simulink library "pne_pne3d_generic_std"  (R2016a)
(part 6 of 7)

p510 "pne_brk_PowerBoost_massfracH2O (init) export=true name=pne_brk_PowerBoost_massfracH2O prio=1 dataSetName=std dataClassType=initIO dataClassName=initIO unit='-' description='pne_brk_PowerBoost_massfracH2O (init)': IO_PNE_Generic.pne_brk_PowerBoost_massfracH2O_0 [-]"; p511 "pne_brk_PowerBoost_mdot (init) export=true name=pne_brk_PowerBoost_mdot prio=1 dataSetName=std dataClassType=initIO dataClassName=initIO unit=kg/s description='pne_brk_PowerBoost_mdot': IO_PNE_Generic.pne_brk_PowerBoost_mdot_0 [-]"; p512 "pne_brk_PowerBoost_pressure [mbar] (init) export=true name=pne_brk_PowerBoost_pressure prio=1 dataSetName=std dataClassType=initIO dataClassName=initIO unit=mbar description='pne_brk_PowerBoost_pressure [mbar] (init)': IO_PNE_Generic.pne_brk_PowerBoost_pressure_0 [-]"; p513 "pne_brk_PowerBoost_Temperature [degC] (init) export=true name=pne_brk_PowerBoost_Temperature prio=1 dataSetName=std dataClassType=initIO dataClassName=initIO unit=degC description='pne_brk_PowerBoost_Temperature [degC] (init)': IO_PNE_Generic.pne_brk_PowerBoost_Temperature_0 [-]"; p514 "Parking Brake Pressure [bar] (init) export=true name=pne_brk_pRelPkBrk prio=1 dataSetName=std dataClassType=initIO dataClassName=initIO unit=bar description='Parking Brake Pressure [bar] (init)': IO_PNE_Generic.pne_brk_pRelPkBrk_0 [-]"; p515 "pne_brk_RearAxle_left_pAct (init) export=true name=pne_brk_RearAxle_left_pAct prio=1 dataSetName=std dataClassType=initIO dataClassName=initIO unit=bar description='pne_brk_RearAxle_left_pAct (init)': IO_PNE_Generic.pne_brk_RearAxle_left_pAct_0 [-]"; p516 "pne_brk_RearAxle_left_rotVel (init) export=true name=pne_brk_RearAxle_left_rotVel prio=1 dataSetName=std dataClassType=initIO dataClassName=initIO unit=rad/s description='pne_brk_RearAxle_left_rotVel (init)': IO_PNE_Generic.pne_brk_RearAxle_left_rotVel_0 [-]"; p517 "pne_brk_RearAxle_right_pAct (init) export=true name=pne_brk_RearAxle_right_pAct prio=1 dataSetName=std dataClassType=initIO dataClassName=initIO unit=bar description='pne_brk_RearAxle_right_pAct (init)': IO_PNE_Generic.pne_brk_RearAxle_right_pAct_0 [-]"; p518 "pne_brk_RearAxle_right_rotVel (init) export=true name=pne_brk_RearAxle_right_rotVel prio=1 dataSetName=std dataClassType=initIO dataClassName=initIO unit=rad/s description='pne_brk_RearAxle_right_rotVel (init)': IO_PNE_Generic.pne_brk_RearAxle_right_rotVel_0 [-]"; p519 "pne_brk_reg_active (init), Regeneraaton active export=true name=pne_brk_reg_active prio=1 dataSetName=std dataClassType=initIO dataClassName=initIO unit='-' description='Regeneraaton active': IO_PNE_Generic.pne_brk_reg_active_0 [-]"; p520 "wheel speed addional left wheel (init) export=true name=pne_brk_rotVel_al prio=1 dataSetName=std dataClassType=initIO dataClassName=initIO unit=rad/s description='wheel speed addional left wheel (init)': IO_PNE_Generic.pne_brk_rotVel_al_0 [-]"; p521 "wheel speed additional right wheel (init) export=true name=pne_brk_rotVel_ar prio=1 dataSetName=std dataClassType=initIO dataClassName=initIO unit=rad/s description='wheel speed additional right wheel (init)': IO_PNE_Generic.pne_brk_rotVel_ar_0 [-]"; p522 "wheel speed front left wheel (init) export=true name=pne_brk_rotVel_fl prio=1 dataSetName=std dataClassType=initIO dataClassName=initIO unit=rad/s description='wheel speed front left wheel (init)': IO_PNE_Generic.pne_brk_rotVel_fl_0 [-]"; p523 "wheel speed front right wheel (init) export=true name=pne_brk_rotVel_fr prio=1 dataSetName=std dataClassType=initIO dataClassName=initIO unit=rad/s description='wheel speed front right wheel (init)': IO_PNE_Generic.pne_brk_rotVel_fr_0 [-]"; p524 "wheel speed rear left wheel (init) export=true name=pne_brk_rotVel_rl prio=1 dataSetName=std dataClassType=initIO dataClassName=initIO unit=rad/s description='wheel speed rear left wheel (init)': IO_PNE_Generic.pne_brk_rotVel_rl_0 [-]"; p525 "wheel speed rear right wheel (init) export=true name=pne_brk_rotVel_rr prio=1 dataSetName=std dataClassType=initIO dataClassName=initIO unit=rad/s description='wheel speed rear right wheel (init)': IO_PNE_Generic.pne_brk_rotVel_rr_0 [-]"; p526 "wheel speed trailer axle1 left wheel (init) export=true name=pne_brk_rotVel_t1l prio=1 dataSetName=std dataClassType=initIO dataClassName=initIO unit=rad/s description='wheel speed trailer axle1 left wheel (init)': IO_PNE_Generic.pne_brk_rotVel_t1l_0 [-]"; p527 "wheel speed trailer axle1 right wheel (init) export=true name=pne_brk_rotVel_t1r prio=1 dataSetName=std dataClassType=initIO dataClassName=initIO unit=rad/s description='wheel speed trailer axle1 right wheel (init)': IO_PNE_Generic.pne_brk_rotVel_t1r_0 [-]"; p528 "wheel speed trailer axle2 left wheel (init) export=true name=pne_brk_rotVel_t2l prio=1 dataSetName=std dataClassType=initIO dataClassName=initIO unit=rad/s description='wheel speed trailer axle2 left wheel (init)': IO_PNE_Generic.pne_brk_rotVel_t2l_0 [-]"; p529 "wheel speed trailer axle2 right wheel (init) export=true name=pne_brk_rotVel_t2r prio=1 dataSetName=std dataClassType=initIO dataClassName=initIO unit=rad/s description='wheel speed trailer axle2 right wheel (init)': IO_PNE_Generic.pne_brk_rotVel_t2r_0 [-]"; p530 "wheel speed trailer axle3 left wheel (init) export=true name=pne_brk_rotVel_t3l prio=1 dataSetName=std dataClassType=initIO dataClassName=initIO unit=rad/s description='wheel speed trailer axle3 left wheel (init)': IO_PNE_Generic.pne_brk_rotVel_t3l_0 [-]"; p531 "wheel speed trailer axle3 right wheel (init) export=true name=pne_brk_rotVel_t3r prio=1 dataSetName=std dataClassType=initIO dataClassName=initIO unit=rad/s description='wheel speed trailer axle3 right wheel (init)': IO_PNE_Generic.pne_brk_rotVel_t3r_0 [-]"; p532 "pne_brk_TCV_pAct (init) export=true name=pne_brk_TCV_pAct prio=1 dataSetName=std dataClassType=initIO dataClassName=initIO unit=bar description='pne_brk_TCV_pAct (init)': IO_PNE_Generic.pne_brk_TCV_pAct_0 [-]"; p533 "pne_brk_Trailer_RV_Front_pAct (init) export=true name=pne_brk_Trailer_RV_Front_pAct prio=1 dataSetName=std dataClassType=initIO dataClassName=initIO unit=bar description='pne_brk_Trailer_RV_Front_pAct (init)': IO_PNE_Generic.pne_brk_Trailer_RV_Front_pAct_0 [-]"; p534 "pne_brk_Trailer_RV_Rear_pAct (init) export=true name=pne_brk_Trailer_RV_Rear_pAct prio=1 dataSetName=std dataClassType=initIO dataClassName=initIO unit=bar description='pne_brk_Trailer_RV_Rear_pAct (init)': IO_PNE_Generic.pne_brk_Trailer_RV_Rear_pAct_0 [-]"; p535 "pne_brk_TrailerAxle1_BrakingForce_at8p5bar [N] (init) export=true name=pne_brk_TrailerAxle1_BrakingForce_at8p5bar prio=1 dataSetName=std dataClassType=initIO dataClassName=initIO unit=N description='pne_brk_TrailerAxle1_BrakingForce_at8p5bar [N] (init)': IO_PNE_Generic.pne_brk_TrailerAxle1_BrakingForce_at8p5bar_0 [-]"; p536 "pne_brk_TrailerAxle1_BrakingPower [kW] (init) export=true name=pne_brk_TrailerAxle1_BrakingPower prio=1 dataSetName=std dataClassType=initIO dataClassName=initIO unit=kW description='pne_brk_TrailerAxle1_BrakingPower [kW] (init)': IO_PNE_Generic.pne_brk_TrailerAxle1_BrakingPower_0 [-]"; p537 "TrailerAxle 1 left - angular acceleration (init) export=true name=pne_brk_TrailerAxle1_left_angAcc prio=1 dataSetName=std dataClassType=initIO dataClassName=initIO unit=rad/s^2 description='TrailerAxle 1 left - angular acceleration (init)': IO_PNE_Generic.pne_brk_TrailerAxle1_left_angAcc_0 [-]"; p538 "Axle 1 left - angular position (init) export=true name=pne_brk_TrailerAxle1_left_angPos prio=1 dataSetName=std dataClassType=initIO dataClassName=initIO unit=bar description='TrailerAxle 1 left - angular position (init)': IO_PNE_Generic.pne_brk_TrailerAxle1_left_angPos_0 [-]"; p539 "Axle 1 left - angular velocity (init) export=true name=pne_brk_TrailerAxle1_left_angVel prio=1 dataSetName=std dataClassType=initIO dataClassName=initIO unit=rad/s description='TrailerAxle 1 left - angular velocity (init)': IO_PNE_Generic.pne_brk_TrailerAxle1_left_angVel_0 [-]"; p540 "brake correction coefficient kvT trailer axle 1 left (init) export=true name=pne_brk_TrailerAxle1_left_kvT prio=1 dataSetName=std dataClassType=initIO dataClassName=initIO unit='-' description='brake correction coefficient kvT trailer axle 1 left (init)': IO_PNE_Generic.pne_brk_TrailerAxle1_left_kvT_0 [-]"; p541 "brake pad thickness trailer axle 1 left (init) export=true name=pne_brk_TrailerAxle1_left_sPad_sum prio=1 dataSetName=std dataClassType=initIO dataClassName=initIO unit=m description='brake pad thickness trailer axle 1 left (init)': IO_PNE_Generic.pne_brk_TrailerAxle1_left_sPad_sum_0 [-]"; p542 "trailer axle 1 left temperature of the cooling surface area [degC] (init) export=true name=pne_brk_TrailerAxle1_left_Tcooldown prio=1 dataSetName=std dataClassType=initIO dataClassName=initIO unit=degC description='trailer axle 1 left temperature of the cooling surface area [degC] (init)': IO_PNE_Generic.pne_brk_TrailerAxle1_left_Tcooldown_0 [-]"; p543 "trailer axle 1 left temperature of the friction area [degC] (init) export=true name=pne_brk_TrailerAxle1_left_Tfriction prio=1 dataSetName=std dataClassType=initIO dataClassName=initIO unit=degC description='trailer axle 1 left temperature of the friction area [degC] (init)': IO_PNE_Generic.pne_brk_TrailerAxle1_left_Tfriction_0 [-]"; p544 "trailer axle 1 left temperature of the friction area [degC] (init) export=true name=pne_brk_TrailerAxle1_left_Tinterior prio=1 dataSetName=std dataClassType=initIO dataClassName=initIO unit=degC description='trailer axle 1 left inner temperature [degC] (init)': IO_PNE_Generic.pne_brk_TrailerAxle1_left_Tinterior_0 [-]"; p545 "pne_brk_TrailerAxle1_left_torque [Nm] (init) export=true name=pne_brk_TrailerAxle1_left_torque prio=1 dataSetName=std dataClassType=initIO dataClassName=initIO unit=Nm description='pne_brk_TrailerAxle1_left_torque [Nm] (init)': IO_PNE_Generic.pne_brk_TrailerAxle1_left_torque_0 [-]"; p546 "pne_brk_TrailerAxle1_left_torque_grinding [Nm] (init) export=true name=pne_brk_TrailerAxle1_left_torque_grinding prio=1 dataSetName=std dataClassType=initIO dataClassName=initIO unit=Nm description='pne_brk_TrailerAxle1_left_torque_grinding [Nm] (init)': IO_PNE_Generic.pne_brk_TrailerAxle1_left_torque_grinding_0 [-]"; p547 "TrailerAxle 1 right - angular acceleration (init) export=true name=pne_brk_TrailerAxle1_right_angAcc prio=1 dataSetName=std dataClassType=initIO dataClassName=initIO unit=rad/s^2 description='TrailerAxle 1 right - angular acceleration (init)': IO_PNE_Generic.pne_brk_TrailerAxle1_right_angAcc_0 [-]"; p548 "Axle 1 right - angular position (init) export=true name=pne_brk_TrailerAxle1_right_angPos prio=1 dataSetName=std dataClassType=initIO dataClassName=initIO unit=bar description='TrailerAxle 1 right - angular position (init)': IO_PNE_Generic.pne_brk_TrailerAxle1_right_angPos_0 [-]"; p549 "Axle 1 right - angular velocity (init) export=true name=pne_brk_TrailerAxle1_right_angVel prio=1 dataSetName=std dataClassType=initIO dataClassName=initIO unit=rad/s description='TrailerAxle 1 right - angular velocity (init)': IO_PNE_Generic.pne_brk_TrailerAxle1_right_angVel_0 [-]"; p550 "brake correction coefficient kvT trailer axle 1 right (init) export=true name=pne_brk_TrailerAxle1_right_kvT prio=1 dataSetName=std dataClassType=initIO dataClassName=initIO unit='-' description='brake correction coefficient kvT trailer axle 1 right (init)': IO_PNE_Generic.pne_brk_TrailerAxle1_right_kvT_0 [-]"; p551 "brake pad thickness trailer axle 1 right (init) export=true name=pne_brk_TrailerAxle1_right_sPad_sum prio=1 dataSetName=std dataClassType=initIO dataClassName=initIO unit=m description='brake pad thickness trailer axle 1 right (init)': IO_PNE_Generic.pne_brk_TrailerAxle1_right_sPad_sum_0 [-]"; p552 "trailer axle 1 right temperature of the cooling surface area [degC] (init) export=true name=pne_brk_TrailerAxle1_right_Tcooldown prio=1 dataSetName=std dataClassType=initIO dataClassName=initIO unit=degC description='trailer axle 1 right temperature of the cooling surface area [degC] (init)': IO_PNE_Generic.pne_brk_TrailerAxle1_right_Tcooldown_0 [-]"; p553 "trailer axle 1 right temperature of the friction area [degC] (init) export=true name=pne_brk_TrailerAxle1_right_Tfriction prio=1 dataSetName=std dataClassType=initIO dataClassName=initIO unit=degC description='trailer axle 1 right temperature of the friction area [degC] (init)': IO_PNE_Generic.pne_brk_TrailerAxle1_right_Tfriction_0 [-]"; p554 "trailer axle 1 right temperature of the friction area [degC] (init) export=true name=pne_brk_TrailerAxle1_right_Tinterior prio=1 dataSetName=std dataClassType=initIO dataClassName=initIO unit=degC description='trailer axle 1 right inner temperature [degC] (init)': IO_PNE_Generic.pne_brk_TrailerAxle1_right_Tinterior_0 [-]"; p555 "pne_brk_TrailerAxle1_right_torque [Nm] (init) export=true name=pne_brk_TrailerAxle1_right_torque prio=1 dataSetName=std dataClassType=initIO dataClassName=initIO unit=Nm description='pne_brk_TrailerAxle1_right_torque [Nm] (init)': IO_PNE_Generic.pne_brk_TrailerAxle1_right_torque_0 [-]"; p556 "pne_brk_TrailerAxle1_right_torque_grinding [Nm] (init) export=true name=pne_brk_TrailerAxle1_right_torque_grinding prio=1 dataSetName=std dataClassType=initIO dataClassName=initIO unit=Nm description='pne_brk_TrailerAxle1_right_torque_grinding [Nm] (init)': IO_PNE_Generic.pne_brk_TrailerAxle1_right_torque_grinding_0 [-]"; p557 "pne_brk_TrailerAxle1_torque_sns [Nm] (init) export=true name=pne_brk_TrailerAxle1_torque_sns prio=1 dataSetName=std dataClassType=initIO dataClassName=initIO unit=Nm description='pne_brk_TrailerAxle1_torque_sns [Nm] (init)': IO_PNE_Generic.pne_brk_TrailerAxle1_torque_sns_0 [-]"; p558 "Cylinder Force Trailer Brake Cylinder1 [N] (init) export=true name=pne_brk_TrailerAxle1Brake_Fcyl prio=1 dataSetName=std dataClassType=initIO dataClassName=initIO unit=N description='Cylinder Force Trailer Brake Cylinder1 [N] (init)': IO_PNE_Generic.pne_brk_TrailerAxle1Brake_Fcyl_0 [-]"; p559 "Pressure (relative) Trailer Brake Cylinder1 left [bar] (init) export=true name=pne_brk_TrailerAxle1Brake_left_pRel prio=1 dataSetName=std dataClassType=initIO dataClassName=initIO unit=bar description='Pressure (relative) Trailer Brake Cylinder1 left [bar] (init)': IO_PNE_Generic.pne_brk_TrailerAxle1Brake_left_pRel_0 [-]"; p560 "Pressure (relative) Trailer Brake Cylinder1 right [bar] (init) export=true name=pne_brk_TrailerAxle1Brake_right_pRel prio=1 dataSetName=std dataClassType=initIO dataClassName=initIO unit=bar description='Pressure (relative) Trailer Brake Cylinder1 right [bar] (init)': IO_PNE_Generic.pne_brk_TrailerAxle1Brake_right_pRel_0 [-]"; p561 "Piston Stroke Trailer Brake Cylinder1 [mm] (init) export=true name=pne_brk_TrailerAxle1Brake_stroke prio=1 dataSetName=std dataClassType=initIO dataClassName=initIO unit=mm description='Piston Stroke Trailer Brake Cylinder1 [mm] (init)': IO_PNE_Generic.pne_brk_TrailerAxle1Brake_stroke_0 [-]"; p562 "pne_brk_TrailerAxle1Brake_Vol [dm3] (init) export=true name=pne_brk_TrailerAxle1Brake_Vol prio=1 dataSetName=std dataClassType=initIO dataClassName=initIO unit=l description='pne_brk_TrailerAxle1Brake_Vol [dm3] (init)': IO_PNE_Generic.pne_brk_TrailerAxle1Brake_Vol_0 [-]"; p563 "pne_brk_TrailerAxle2_BrakingForce_at8p5bar [N] (init) export=true name=pne_brk_TrailerAxle2_BrakingForce_at8p5bar prio=1 dataSetName=std dataClassType=initIO dataClassName=initIO unit=N description='pne_brk_TrailerAxle2_BrakingForce_at8p5bar [N] (init)': IO_PNE_Generic.pne_brk_TrailerAxle2_BrakingForce_at8p5bar_0 [-]"; p564 "pne_brk_TrailerAxle2_BrakingPower [kW] (init) export=true name=pne_brk_TrailerAxle2_BrakingPower prio=1 dataSetName=std dataClassType=initIO dataClassName=initIO unit=kW description='pne_brk_TrailerAxle2_BrakingPower [kW] (init)': IO_PNE_Generic.pne_brk_TrailerAxle2_BrakingPower_0 [-]"; p565 "TrailerAxle 2 left - angular acceleration (init) export=true name=pne_brk_TrailerAxle2_left_angAcc prio=1 dataSetName=std dataClassType=initIO dataClassName=initIO unit=rad/s^2 description='TrailerAxle 2 left - angular acceleration (init)': IO_PNE_Generic.pne_brk_TrailerAxle2_left_angAcc_0 [-]"; p566 "TrailerAxle 2 left - angular position (init) export=true name=pne_brk_TrailerAxle2_left_angPos prio=1 dataSetName=std dataClassType=initIO dataClassName=initIO unit=bar description='TrailerAxle 2 left - angular position (init)': IO_PNE_Generic.pne_brk_TrailerAxle2_left_angPos_0 [-]"; p567 "TrailerAxle 2 left - angular velocity (init) export=true name=pne_brk_TrailerAxle2_left_angVel prio=1 dataSetName=std dataClassType=initIO dataClassName=initIO unit=rad/s description='TrailerAxle 2 left - angular velocity (init)': IO_PNE_Generic.pne_brk_TrailerAxle2_left_angVel_0 [-]"; p568 "brake correction coefficient kvT trailer axle 2 left (init) export=true name=pne_brk_TrailerAxle2_left_kvT prio=1 dataSetName=std dataClassType=initIO dataClassName=initIO unit='-' description='brake correction coefficient kvT trailer axle 2 left (init)': IO_PNE_Generic.pne_brk_TrailerAxle2_left_kvT_0 [-]"; p569 "brake pad thickness trailer axle 2 left (init) export=true name=pne_brk_TrailerAxle2_left_sPad_sum prio=1 dataSetName=std dataClassType=initIO dataClassName=initIO unit=m description='brake pad thickness trailer axle 2 left (init)': IO_PNE_Generic.pne_brk_TrailerAxle2_left_sPad_sum_0 [-]"; p570 "trailer axle 2 left temperature of the cooling surface area [degC] (init) export=true name=pne_brk_TrailerAxle2_left_Tcooldown prio=1 dataSetName=std dataClassType=initIO dataClassName=initIO unit=degC description='trailer axle 2 left temperature of the cooling surface area [degC] (init)': IO_PNE_Generic.pne_brk_TrailerAxle2_left_Tcooldown_0 [-]"; p571 "trailer axle 2 left temperature of the friction area [degC] (init) export=true name=pne_brk_TrailerAxle2_left_Tfriction prio=1 dataSetName=std dataClassType=initIO dataClassName=initIO unit=degC description='trailer axle 2 left temperature of the friction area [degC] (init)': IO_PNE_Generic.pne_brk_TrailerAxle2_left_Tfriction_0 [-]"; p572 "trailer axle 2 left temperature of the friction area [degC] (init) export=true name=pne_brk_TrailerAxle2_left_Tinterior prio=1 dataSetName=std dataClassType=initIO dataClassName=initIO unit=degC description='trailer axle 2 left inner temperature [degC] (init)': IO_PNE_Generic.pne_brk_TrailerAxle2_left_Tinterior_0 [-]"; p573 "pne_brk_TrailerAxle2_left_torque [Nm] (init) export=true name=pne_brk_TrailerAxle2_left_torque prio=1 dataSetName=std dataClassType=initIO dataClassName=initIO unit=Nm description='pne_brk_TrailerAxle2_left_torque [Nm] (init)': IO_PNE_Generic.pne_brk_TrailerAxle2_left_torque_0 [-]"; p574 "pne_brk_TrailerAxle2_left_torque_grinding [Nm] (init) export=true name=pne_brk_TrailerAxle2_left_torque_grinding prio=1 dataSetName=std dataClassType=initIO dataClassName=initIO unit=Nm description='pne_brk_TrailerAxle2_left_torque_grinding [Nm] (init)': IO_PNE_Generic.pne_brk_TrailerAxle2_left_torque_grinding_0 [-]"; p575 "TrailerAxle 2 right - angular acceleration (init) export=true name=pne_brk_TrailerAxle2_right_angAcc prio=1 dataSetName=std dataClassType=initIO dataClassName=initIO unit=rad/s^2 description='TrailerAxle 2 right - angular acceleration (init)': IO_PNE_Generic.pne_brk_TrailerAxle2_right_angAcc_0 [-]"; p576 "TrailerAxle 2 right - angular position (init) export=true name=pne_brk_TrailerAxle2_right_angPos prio=1 dataSetName=std dataClassType=initIO dataClassName=initIO unit=bar description='TrailerAxle 2 right - angular position (init)': IO_PNE_Generic.pne_brk_TrailerAxle2_right_angPos_0 [-]"; p577 "TrailerAxle 2 right - angular velocity (init) export=true name=pne_brk_TrailerAxle2_right_angVel prio=1 dataSetName=std dataClassType=initIO dataClassName=initIO unit=rad/s description='TrailerAxle 2 right - angular velocity (init)': IO_PNE_Generic.pne_brk_TrailerAxle2_right_angVel_0 [-]"; p578 "brake correction coefficient kvT trailer axle 2 right (init) export=true name=pne_brk_TrailerAxle2_right_kvT prio=1 dataSetName=std dataClassType=initIO dataClassName=initIO unit='-' description='brake correction coefficient kvT trailer axle 2 right (init)': IO_PNE_Generic.pne_brk_TrailerAxle2_right_kvT_0 [-]"; p579 "brake pad thickness trailer axle 2 right (init) export=true name=pne_brk_TrailerAxle2_right_sPad_sum prio=1 dataSetName=std dataClassType=initIO dataClassName=initIO unit=m description='brake pad thickness trailer axle 2 right (init)': IO_PNE_Generic.pne_brk_TrailerAxle2_right_sPad_sum_0 [-]"; p580 "trailer axle 2 right temperature of the cooling surface area [degC] (init) export=true name=pne_brk_TrailerAxle2_right_Tcooldown prio=1 dataSetName=std dataClassType=initIO dataClassName=initIO unit=degC description='trailer axle 2 right temperature of the cooling surface area [degC] (init)': IO_PNE_Generic.pne_brk_TrailerAxle2_right_Tcooldown_0 [-]"; p581 "trailer axle 2 right temperature of the friction area [degC] (init) export=true name=pne_brk_TrailerAxle2_right_Tfriction prio=1 dataSetName=std dataClassType=initIO dataClassName=initIO unit=degC description='trailer axle 2 right temperature of the friction area [degC] (init)': IO_PNE_Generic.pne_brk_TrailerAxle2_right_Tfriction_0 [-]"; p582 "trailer axle 2 right temperature of the friction area [degC] (init) export=true name=pne_brk_TrailerAxle2_right_Tinterior prio=1 dataSetName=std dataClassType=initIO dataClassName=initIO unit=degC description='trailer axle 2 right inner temperature [degC] (init)': IO_PNE_Generic.pne_brk_TrailerAxle2_right_Tinterior_0 [-]"; p583 "pne_brk_TrailerAxle2_right_torque [Nm] (init) export=true name=pne_brk_TrailerAxle2_right_torque prio=1 dataSetName=std dataClassType=initIO dataClassName=initIO unit=Nm description='pne_brk_TrailerAxle2_right_torque [Nm] (init)': IO_PNE_Generic.pne_brk_TrailerAxle2_right_torque_0 [-]"; p584 "pne_brk_TrailerAxle2_right_torque_grinding [Nm] (init) export=true name=pne_brk_TrailerAxle2_right_torque_grinding prio=1 dataSetName=std dataClassType=initIO dataClassName=initIO unit=Nm description='pne_brk_TrailerAxle2_right_torque_grinding [Nm] (init)': IO_PNE_Generic.pne_brk_TrailerAxle2_right_torque_grinding_0 [-]"; p585 "pne_brk_TrailerAxle2_torque_sns [Nm] (init) export=true name=pne_brk_TrailerAxle2_torque_sns prio=1 dataSetName=std dataClassType=initIO dataClassName=initIO unit=Nm description='pne_brk_TrailerAxle2_torque_sns [Nm] (init)': IO_PNE_Generic.pne_brk_TrailerAxle2_torque_sns_0 [-]"; p586 "Cylinder Force Trailer Brake Cylinder2 [N] (init) export=true name=pne_brk_TrailerAxle2Brake_Fcyl prio=1 dataSetName=std dataClassType=initIO dataClassName=initIO unit=N description='Cylinder Force Trailer Brake Cylinder2 [N] (init)': IO_PNE_Generic.pne_brk_TrailerAxle2Brake_Fcyl_0 [-]"; p587 "Pressure (relative) Trailer Brake Cylinder2 left [bar] (init) export=true name=pne_brk_TrailerAxle2Brake_left_pRel prio=1 dataSetName=std dataClassType=initIO dataClassName=initIO unit=bar description='Pressure (relative) Trailer Brake Cylinder2 left [bar] (init)': IO_PNE_Generic.pne_brk_TrailerAxle2Brake_left_pRel_0 [-]"; p588 "Pressure (relative) Trailer Brake Cylinder2 right [bar] (init) export=true name=pne_brk_TrailerAxle2Brake_right_pRel prio=1 dataSetName=std dataClassType=initIO dataClassName=initIO unit=bar description='Pressure (relative) Trailer Brake Cylinder2 right [bar] (init)': IO_PNE_Generic.pne_brk_TrailerAxle2Brake_right_pRel_0 [-]"; p589 "Piston Stroke Trailer Brake Cylinder2 [mm] (init) export=true name=pne_brk_TrailerAxle2Brake_stroke prio=1 dataSetName=std dataClassType=initIO dataClassName=initIO unit=mm description='Piston Stroke Trailer Brake Cylinder2 [mm] (init)': IO_PNE_Generic.pne_brk_TrailerAxle2Brake_stroke_0 [-]"; p590 "pne_brk_TrailerAxle2Brake_Vol [dm3] (init) export=true name=pne_brk_TrailerAxle2Brake_Vol prio=1 dataSetName=std dataClassType=initIO dataClassName=initIO unit=l description='pne_brk_TrailerAxle2Brake_Vol [dm3] (init)': IO_PNE_Generic.pne_brk_TrailerAxle2Brake_Vol_0 [-]"; p591 "pne_brk_TrailerAxle3_BrakingForce_at8p5bar [N] (init) export=true name=pne_brk_TrailerAxle3_BrakingForce_at8p5bar prio=1 dataSetName=std dataClassType=initIO dataClassName=initIO unit=N description='pne_brk_TrailerAxle3_BrakingForce_at8p5bar [N] (init)': IO_PNE_Generic.pne_brk_TrailerAxle3_BrakingForce_at8p5bar_0 [-]"; p592 "pne_brk_TrailerAxle3_BrakingPower [kW] (init) export=true name=pne_brk_TrailerAxle3_BrakingPower prio=1 dataSetName=std dataClassType=initIO dataClassName=initIO unit=kW description='pne_brk_TrailerAxle3_BrakingPower [kW] (init)': IO_PNE_Generic.pne_brk_TrailerAxle3_BrakingPower_0 [-]"; p593 "TrailerAxle 3 left - angular acceleration (init) export=true name=pne_brk_TrailerAxle3_left_angAcc prio=1 dataSetName=std dataClassType=initIO dataClassName=initIO unit=rad/s^2 description='TrailerAxle 3 left - angular acceleration (init)': IO_PNE_Generic.pne_brk_TrailerAxle3_left_angAcc_0 [-]"; p594 "TrailerAxle 3 left - angular position (init) export=true name=pne_brk_TrailerAxle3_left_angPos prio=1 dataSetName=std dataClassType=initIO dataClassName=initIO unit=bar description='TrailerAxle 3 left - angular position (init)': IO_PNE_Generic.pne_brk_TrailerAxle3_left_angPos_0 [-]"; p595 "TrailerAxle 3 left - angular velocity (init) export=true name=pne_brk_TrailerAxle3_left_angVel prio=1 dataSetName=std dataClassType=initIO dataClassName=initIO unit=rad/s description='TrailerAxle 3 left - angular velocity (init)': IO_PNE_Generic.pne_brk_TrailerAxle3_left_angVel_0 [-]"; p596 "brake correction coefficient kvT trailer axle 3 left (init) export=true name=pne_brk_TrailerAxle3_left_kvT prio=1 dataSetName=std dataClassType=initIO dataClassName=initIO unit='-' description='brake correction coefficient kvT trailer axle 3 left (init)': IO_PNE_Generic.pne_brk_TrailerAxle3_left_kvT_0 [-]"; p597 "brake pad thickness trailer axle 3 left (init) export=true name=pne_brk_TrailerAxle3_left_sPad_sum prio=1 dataSetName=std dataClassType=initIO dataClassName=initIO unit=m description='brake pad thickness trailer axle 3 left (init)': IO_PNE_Generic.pne_brk_TrailerAxle3_left_sPad_sum_0 [-]"; p598 "trailer axle 3 left temperature of the cooling surface area [degC] (init) export=true name=pne_brk_TrailerAxle3_left_Tcooldown prio=1 dataSetName=std dataClassType=initIO dataClassName=initIO unit=degC description='trailer axle 3 left temperature of the cooling surface area [degC] (init)': IO_PNE_Generic.pne_brk_TrailerAxle3_left_Tcooldown_0 [-]"; p599 "trailer axle 3 left temperature of the friction area [degC] (init) export=true name=pne_brk_TrailerAxle3_left_Tfriction prio=1 dataSetName=std dataClassType=initIO dataClassName=initIO unit=degC description='trailer axle 3 left temperature of the friction area [degC] (init)': IO_PNE_Generic.pne_brk_TrailerAxle3_left_Tfriction_0 [-]"; p600 "trailer axle 3 left temperature of the friction area [degC] (init) export=true name=pne_brk_TrailerAxle3_left_Tinterior prio=1 dataSetName=std dataClassType=initIO dataClassName=initIO unit=degC description='trailer axle 3 left inner temperature [degC] (init)': IO_PNE_Generic.pne_brk_TrailerAxle3_left_Tinterior_0 [-]"; p601 "pne_brk_TrailerAxle3_left_torque [Nm] (init) export=true name=pne_brk_TrailerAxle3_left_torque prio=1 dataSetName=std dataClassType=initIO dataClassName=initIO unit=Nm description='pne_brk_TrailerAxle3_left_torque [Nm] (init)': IO_PNE_Generic.pne_brk_TrailerAxle3_left_torque_0 [-]"; p602 "pne_brk_TrailerAxle3_left_torque_grinding [Nm] (init) export=true name=pne_brk_TrailerAxle3_left_torque_grinding prio=1 dataSetName=std dataClassType=initIO dataClassName=initIO unit=Nm description='pne_brk_TrailerAxle3_left_torque_grinding [Nm] (init)': IO_PNE_Generic.pne_brk_TrailerAxle3_left_torque_grinding_0 [-]"; p603 "TrailerAxle 3 right - angular acceleration (init) export=true name=pne_brk_TrailerAxle3_right_angAcc prio=1 dataSetName=std dataClassType=initIO dataClassName=initIO unit=rad/s^2 description='TrailerAxle 3 right - angular acceleration (init)': IO_PNE_Generic.pne_brk_TrailerAxle3_right_angAcc_0 [-]"; p604 "TrailerAxle 3 right - angular position (init) export=true name=pne_brk_TrailerAxle3_right_angPos prio=1 dataSetName=std dataClassType=initIO dataClassName=initIO unit=bar description='TrailerAxle 3 right - angular position (init)': IO_PNE_Generic.pne_brk_TrailerAxle3_right_angPos_0 [-]"; p605 "TrailerAxle 3 right - angular velocity (init) export=true name=pne_brk_TrailerAxle3_right_angVel prio=1 dataSetName=std dataClassType=initIO dataClassName=initIO unit=rad/s description='TrailerAxle 3 right - angular velocity (init)': IO_PNE_Generic.pne_brk_TrailerAxle3_right_angVel_0 [-]"; p606 "brake correction coefficient kvT trailer axle 3 right (init) export=true name=pne_brk_TrailerAxle3_right_kvT prio=1 dataSetName=std dataClassType=initIO dataClassName=initIO unit='-' description='brake correction coefficient kvT trailer axle 3 right (init)': IO_PNE_Generic.pne_brk_TrailerAxle3_right_kvT_0 [-]"; p607 "brake pad thickness trailer axle 3 right (init) export=true name=pne_brk_TrailerAxle3_right_sPad_sum prio=1 dataSetName=std dataClassType=initIO dataClassName=initIO unit=m description='brake pad thickness trailer axle 3 right (init)': IO_PNE_Generic.pne_brk_TrailerAxle3_right_sPad_sum_0 [-]"; p608 "trailer axle 3 right temperature of the cooling surface area [degC] (init) export=true name=pne_brk_TrailerAxle3_right_Tcooldown prio=1 dataSetName=std dataClassType=initIO dataClassName=initIO unit=degC description='trailer axle 3 right temperature of the cooling surface area [degC] (init)': IO_PNE_Generic.pne_brk_TrailerAxle3_right_Tcooldown_0 [-]"; p609 "trailer axle 3 right temperature of the friction area [degC] (init) export=true name=pne_brk_TrailerAxle3_right_Tfriction prio=1 dataSetName=std dataClassType=initIO dataClassName=initIO unit=degC description='trailer axle 3 right temperature of the friction area [degC] (init)': IO_PNE_Generic.pne_brk_TrailerAxle3_right_Tfriction_0 [-]"; p610 "trailer axle 3 right temperature of the friction area [degC] (init) export=true name=pne_brk_TrailerAxle3_right_Tinterior prio=1 dataSetName=std dataClassType=initIO dataClassName=initIO unit=degC description='trailer axle 3 right inner temperature [degC] (init)': IO_PNE_Generic.pne_brk_TrailerAxle3_right_Tinterior_0 [-]"; p611 "pne_brk_TrailerAxle3_right_torque [Nm] (init) export=true name=pne_brk_TrailerAxle3_right_torque prio=1 dataSetName=std dataClassType=initIO dataClassName=initIO unit=Nm description='pne_brk_TrailerAxle3_right_torque [Nm] (init)': IO_PNE_Generic.pne_brk_TrailerAxle3_right_torque_0 [-]"; p612 "pne_brk_TrailerAxle3_right_torque_grinding [Nm] (init) export=true name=pne_brk_TrailerAxle3_right_torque_grinding prio=1 dataSetName=std dataClassType=initIO dataClassName=initIO unit=Nm description='pne_brk_TrailerAxle3_right_torque_grinding [Nm] (init)': IO_PNE_Generic.pne_brk_TrailerAxle3_right_torque_grinding_0 [-]"; p613 "pne_brk_TrailerAxle3_torque_sns [Nm] (init) export=true name=pne_brk_TrailerAxle3_torque_sns prio=1 dataSetName=std dataClassType=initIO dataClassName=initIO unit=Nm description='pne_brk_TrailerAxle3_torque_sns [Nm] (init)': IO_PNE_Generic.pne_brk_TrailerAxle3_torque_sns_0 [-]"; p614 "Cylinder Force Trailer Brake Cylinder3 [N] (init) export=true name=pne_brk_TrailerAxle3Brake_Fcyl prio=1 dataSetName=std dataClassType=initIO dataClassName=initIO unit=N description='Cylinder Force Trailer Brake Cylinder3 [N] (init)': IO_PNE_Generic.pne_brk_TrailerAxle3Brake_Fcyl_0 [-]"; p615 "Pressure (relative) Trailer Brake Cylinder3 left [bar] (init) export=true name=pne_brk_TrailerAxle3Brake_left_pRel prio=1 dataSetName=std dataClassType=initIO dataClassName=initIO unit=bar description='Pressure (relative) Trailer Brake Cylinder3 left [bar] (init)': IO_PNE_Generic.pne_brk_TrailerAxle3Brake_left_pRel_0 [-]"; p616 "Pressure (relative) Trailer Brake Cylinder3 right [bar] (init) export=true name=pne_brk_TrailerAxle3Brake_right_pRel prio=1 dataSetName=std dataClassType=initIO dataClassName=initIO unit=bar description='Pressure (relative) Trailer Brake Cylinder3 right [bar] (init)': IO_PNE_Generic.pne_brk_TrailerAxle3Brake_right_pRel_0 [-]"; p617 "Piston Stroke Trailer Brake Cylinder3 [mm] (init) export=true name=pne_brk_TrailerAxle3Brake_stroke prio=1 dataSetName=std dataClassType=initIO dataClassName=initIO unit=mm description='Piston Stroke Trailer Brake Cylinder3 [mm] (init)': IO_PNE_Generic.pne_brk_TrailerAxle3Brake_stroke_0 [-]"; p618 "pne_brk_TrailerAxle3Brake_Vol [dm^3] (init) export=true name=pne_brk_TrailerAxle3Brake_Vol prio=1 dataSetName=std dataClassType=initIO dataClassName=initIO unit=l description='pne_brk_TrailerAxle3Brake_Vol [dm^3] (init)': IO_PNE_Generic.pne_brk_TrailerAxle3Brake_Vol_0 [-]"; p619 "Relative Pressure Tank1 [bar] (init) export=true name=pne_brk_V1_pRel prio=1 dataSetName=std dataClassType=initIO dataClassName=initIO unit=bar description='Relative Pressure Tank1 [bar] (init) ': IO_PNE_Generic.pne_brk_V1_pRel_0 [-]"; p620 "Temperature Tank1 [degC] (init) export=true name=pne_brk_V1_Temp prio=1 dataSetName=std dataClassType=initIO dataClassName=initIO unit=degC description='Temperature Tank1 [degC] (init)': IO_PNE_Generic.pne_brk_V1_Temp_0 [-]"; p621 "Relative Pressure Tank2 [bar] (init) export=true name=pne_brk_V2_pRel prio=1 dataSetName=std dataClassType=initIO dataClassName=initIO unit=bar description='Relative Pressure Tank2 [bar] (init) ': IO_PNE_Generic.pne_brk_V2_pRel_0 [-]"; p622 "Temperature Tank2 [degC] (init) export=true name=pne_brk_V2_Temp prio=1 dataSetName=std dataClassType=initIO dataClassName=initIO unit=degC description='Temperature Tank2 [degC] (init)': IO_PNE_Generic.pne_brk_V2_Temp_0 [-]"; p623 "Relative Pressure Tank3 [bar] (init) export=true name=pne_brk_V3_pRel prio=1 dataSetName=std dataClassType=initIO dataClassName=initIO unit=bar description='Relative Pressure Tank3 [bar] (init)': IO_PNE_Generic.pne_brk_V3_pRel_0 [-]"; p624 "Temperature Tank3 [degC] (init) export=true name=pne_brk_V3_Temp prio=1 dataSetName=std dataClassType=initIO dataClassName=initIO unit=degC description='Temperature Tank3 [degC] (init)': IO_PNE_Generic.pne_brk_V3_Temp_0 [-]"; p625 "Relative Pressure Tank4 [bar] (init) export=true name=pne_brk_V4_pRel prio=1 dataSetName=std dataClassType=initIO dataClassName=initIO unit=bar description='Relative Pressure Tank4 [bar] (init)': IO_PNE_Generic.pne_brk_V4_pRel_0 [-]"; p626 "Temperature Tank4 [degC] (init) export=true name=pne_brk_V4_Temp prio=1 dataSetName=std dataClassType=initIO dataClassName=initIO unit=degC description='Temperature Tank4 [degC] (init)': IO_PNE_Generic.pne_brk_V4_Temp_0 [-]"; p627 "Relative Pressure Tank5 [bar] (init) export=true name=pne_brk_V5_pRel prio=1 dataSetName=std dataClassType=initIO dataClassName=initIO unit=bar description='Relative Pressure Tank5 [bar] (init)': IO_PNE_Generic.pne_brk_V5_pRel_0 [-]"; p628 "Temperature Tank5 [degC] (init) export=true name=pne_brk_V5_Temp prio=1 dataSetName=std dataClassType=initIO dataClassName=initIO unit=degC description='Temperature Tank5 [degC] (init)': IO_PNE_Generic.pne_brk_V5_Temp_0 [-]"; p629 "Relative Pressure Tank6 [bar] (init) export=true name=pne_brk_V6_pRel prio=1 dataSetName=std dataClassType=initIO dataClassName=initIO unit=bar description='Relative Pressure Tank6 [bar] (init)': IO_PNE_Generic.pne_brk_V6_pRel_0 [-]"; p630 "Temperature Tank6 [degC] (init) export=true name=pne_brk_V6_Temp prio=1 dataSetName=std dataClassType=initIO dataClassName=initIO unit=degC description='Temperature Tank6 [degC] (init)': IO_PNE_Generic.pne_brk_V6_Temp_0 [-]"; p631 "Relative Pressure Tank7 [bar] (init) export=true name=pne_brk_V7_pRel prio=1 dataSetName=std dataClassType=initIO dataClassName=initIO unit=bar description='Relative Pressure Tank7 [bar] (init)': IO_PNE_Generic.pne_brk_V7_pRel_0 [-]"; p632 "Temperature Tank7 [degC] (init) export=true name=pne_brk_V7_Temp prio=1 dataSetName=std dataClassType=initIO dataClassName=initIO unit=degC description='Temperature Tank7 [degC] (init)': IO_PNE_Generic.pne_brk_V7_Temp_0 [-]"; p633 "Relative Pressure Tank8 [bar] (init) export=true name=pne_brk_V8_pRel prio=1 dataSetName=std dataClassType=initIO dataClassName=initIO unit=bar description='Relative Pressure Tank8 [bar] (init)': IO_PNE_Generic.pne_brk_V8_pRel_0 [-]"; p634 "Temperature Tank8 [degC] (init) export=true name=pne_brk_V8_Temp prio=1 dataSetName=std dataClassType=initIO dataClassName=initIO unit=degC description='Temperature Tank8 [degC] (init)': IO_PNE_Generic.pne_brk_V8_Temp_0 [-]"; p635 "Relative Pressure Vsupply Input [bar] (init) export=true name=pne_brk_Vsup_pRel prio=1 dataSetName=std dataClassType=initIO dataClassName=initIO unit=bar description='Relative Pressure Vsupply Input [bar] (init)': IO_PNE_Generic.pne_brk_Vsup_pRel_0 [-]"; p636 "Temperature Vsupply Input [degC] (init) export=true name=pne_brk_Vsup_Temp prio=1 dataSetName=std dataClassType=initIO dataClassName=initIO unit=degC description='Temperature Vsupply Input [degC] (init)': IO_PNE_Generic.pne_brk_Vsup_Temp_0 [-]"; p637 "Relative Pressure Tank Trailer [bar] (init) export=true name=pne_brk_VTrailer_pRel prio=1 dataSetName=std dataClassType=initIO dataClassName=initIO unit=bar description='Relative Pressure Tank Trailer [bar] (init)': IO_PNE_Generic.pne_brk_VTrailer_pRel_0 [-]"; p638 "Temperature Tank Trailer [degC] (init) export=true name=pne_brk_VTrailer_Temp prio=1 dataSetName=std dataClassType=initIO dataClassName=initIO unit=degC description='Temperature Tank Trailer [degC] (init)': IO_PNE_Generic.pne_brk_VTrailer_Temp_0 [-]"; p639 "pne_brk_WetLvl_Cntr (init), Calculated Wettnesslevel of the cartridge / Nl export=true name=pne_brk_WetLvl_Cntr prio=1 dataSetName=std dataClassType=initIO dataClassName=initIO unit='Nl' description='Calculated Wettnesslevel of the cartridge / Nl': IO_PNE_Generic.pne_brk_WetLvl_Cntr_0 [-]"; p640 "pne_susp_A1_Le_Posn (init) export=true name=pne_susp_A1_Le_Posn prio=1 dataSetName=std dataClassType=initIO dataClassName=initIO unit='-' description='pne_susp_A1_Le_Posn (init)': IO_PNE_Generic.pne_susp_A1_Le_Posn_0 [-]"; p641 "pne_susp_A1_Ri_Posn (init) export=true name=pne_susp_A1_Ri_Posn prio=1 dataSetName=std dataClassType=initIO dataClassName=initIO unit='-' description='pne_susp_A1_Ri_Posn (init)': IO_PNE_Generic.pne_susp_A1_Ri_Posn_0 [-]"; p642 "pne_susp_A2_Le_Posn (init) export=true name=pne_susp_A2_Le_Posn prio=1 dataSetName=std dataClassType=initIO dataClassName=initIO unit='-' description='pne_susp_A2_Le_Posn (init)': IO_PNE_Generic.pne_susp_A2_Le_Posn_0 [-]"; p643 "pne_susp_A2_Ri_Posn (init) export=true name=pne_susp_A2_Ri_Posn prio=1 dataSetName=std dataClassType=initIO dataClassName=initIO unit='-' description='pne_susp_A2_Ri_Posn (init)': IO_PNE_Generic.pne_susp_A2_Ri_Posn_0 [-]"; p644 "pne_susp_A3_Le_Posn (init) export=true name=pne_susp_A3_Le_Posn prio=1 dataSetName=std dataClassType=initIO dataClassName=initIO unit='-' description='pne_susp_A3_Le_Posn (init)': IO_PNE_Generic.pne_susp_A3_Le_Posn_0 [-]"; p645 "pne_susp_A3_Ri_Posn (init) export=true name=pne_susp_A3_Ri_Posn prio=1 dataSetName=std dataClassType=initIO dataClassName=initIO unit='-' description='pne_susp_A3_Ri_Posn (init)': IO_PNE_Generic.pne_susp_A3_Ri_Posn_0 [-]"; p646 "pneAux_A1_Le_Rq (init) export=true name=pneAux_A1_Le_Rq prio=1 dataSetName=std dataClassType=initIO dataClassName=initIO unit='-' description='pneAux_A1_Le_Rq': IO_PNE_Generic.pneAux_A1_Le_Rq_0 [-]"; p647 "pneAux_A1_LoLi_Rq (init) export=true name=pneAux_A1_LoLi_Rq prio=1 dataSetName=std dataClassType=initIO dataClassName=initIO unit='-' description='pneAux_A1_LoLi_Rq': IO_PNE_Generic.pneAux_A1_LoLi_Rq_0 [-]"; p648 "pneAux_A1_Ri_Rq (init) export=true name=pneAux_A1_Ri_Rq prio=1 dataSetName=std dataClassType=initIO dataClassName=initIO unit='-' description='pneAux_A1_Ri_Rq': IO_PNE_Generic.pneAux_A1_Ri_Rq_0 [-]"; p649 "pneAux_A2_Le_Rq (init) export=true name=pneAux_A2_Le_Rq prio=1 dataSetName=std dataClassType=initIO dataClassName=initIO unit='-' description='pneAux_A2_Le_Rq': IO_PNE_Generic.pneAux_A2_Le_Rq_0 [-]"; p650 "pneAux_A2_LoLi_Rq (init) export=true name=pneAux_A2_LoLi_Rq prio=1 dataSetName=std dataClassType=initIO dataClassName=initIO unit='-' description='pneAux_A2_LoLi_Rq': IO_PNE_Generic.pneAux_A2_LoLi_Rq_0 [-]"; p651 "pneAux_A2_Ri_Rq (init) export=true name=pneAux_A2_Ri_Rq prio=1 dataSetName=std dataClassType=initIO dataClassName=initIO unit='-' description='pneAux_A2_Ri_Rq': IO_PNE_Generic.pneAux_A2_Ri_Rq_0 [-]"; p652 "pneAux_A3_Le_Rq (init) export=true name=pneAux_A3_Le_Rq prio=1 dataSetName=std dataClassType=initIO dataClassName=initIO unit='-' description='pneAux_A3_Le_Rq': IO_PNE_Generic.pneAux_A3_Le_Rq_0 [-]"; p653 "pneAux_A3_LoLi_Rq (init) export=true name=pneAux_A3_LoLi_Rq prio=1 dataSetName=std dataClassType=initIO dataClassName=initIO unit='-' description='pneAux_A3_LoLi_Rq': IO_PNE_Generic.pneAux_A3_LoLi_Rq_0 [-]"; p654 "pneAux_A3_Ri_Rq (init) export=true name=pneAux_A3_Ri_Rq prio=1 dataSetName=std dataClassType=initIO dataClassName=initIO unit='-' description='pneAux_A3_Ri_Rq (init)': IO_PNE_Generic.pneAux_A3_Ri_Rq_0 [-]"; p655 "pneAux_Axle1_load (init) export=true name=pneAux_Axle1_load prio=1 dataSetName=std dataClassType=initIO dataClassName=initIO unit=kg description='pneAux_Axle1_load': IO_PNE_Generic.pneAux_Axle1_load_0 [-]"; p656 "pneAux_Axle2_load (init) export=true name=pneAux_Axle2_load prio=1 dataSetName=std dataClassType=initIO dataClassName=initIO unit=kg description='pneAux_Axle2_load': IO_PNE_Generic.pneAux_Axle2_load_0 [-]"; p657 "pneAux_Axle3_load (init) export=true name=pneAux_Axle3_load prio=1 dataSetName=std dataClassType=initIO dataClassName=initIO unit=kg description='pneAux_Axle3_load': IO_PNE_Generic.pneAux_Axle3_load_0 [-]"; p658 "pneAux_Axle4_load (init) export=true name=pneAux_Axle4_load prio=1 dataSetName=std dataClassType=initIO dataClassName=initIO unit=kg description='pneAux_Axle4_load': IO_PNE_Generic.pneAux_Axle4_load_0 [-]"; p659 "pneAux_Drs_Rq (init) export=true name=pneAux_Drs_Rq prio=1 dataSetName=std dataClassType=initIO dataClassName=initIO unit='-' description='pneAux_Drs_Rq': IO_PNE_Generic.pneAux_Drs_Rq_0 [-]"; p660 "pneAux_EAPU_overrun (init) export=true name=pneAux_EAPU_overrun prio=1 dataSetName=std dataClassType=initIO dataClassName=initIO unit='-' description='pneAux_EAPU_overrun': IO_PNE_Generic.pneAux_EAPU_overrun_0 [-]"; p661 "pneAux_pSoll_TCV_p43 Trailer Parking Brake (init) export=true name=pneAux_pSoll_TCV_p43 prio=1 dataSetName=std dataClassType=initIO dataClassName=initIO unit=bar description='pneAux_pSoll_TCV_p43 Trailer Parking Brake (init)': IO_PNE_Generic.pneAux_pSoll_TCV_p43_0 [-]"; p662 "Set Pressure Parking Brake (init) export=true name=pneAux_pSollPkBrk prio=1 dataSetName=std dataClassType=initIO dataClassName=initIO unit=bar description='Set Pressure Parking Brake (init)': IO_PNE_Generic.pneAux_pSollPkBrk_0 [-]"; p663 "pneAux_TCV_pDmd_Front_Left (init) export=true name=pneAux_TCV_pDmd_Front_Left prio=1 dataSetName=std dataClassType=initIO dataClassName=initIO unit='-' description='pneAux_TCV_pDmd_Front_Left': IO_PNE_Generic.pneAux_TCV_pDmd_Front_Left_0 [-]"; p664 "pneAux_TCV_pDmd_Front_Right (init) export=true name=pneAux_TCV_pDmd_Front_Right prio=1 dataSetName=std dataClassType=initIO dataClassName=initIO unit='-' description='pneAux_TCV_pDmd_Front_Right': IO_PNE_Generic.pneAux_TCV_pDmd_Front_Right_0 [-]"; p665 "pneAux_TCV_pDmd_Rear_Left (init) export=true name=pneAux_TCV_pDmd_Rear_Left prio=1 dataSetName=std dataClassType=initIO dataClassName=initIO unit='-' description='pneAux_TCV_pDmd_Rear_Left': IO_PNE_Generic.pneAux_TCV_pDmd_Rear_Left_0 [-]"; p666 "pneAux_TCV_pDmd_Rear_Right (init) export=true name=pneAux_TCV_pDmd_Rear_Right prio=1 dataSetName=std dataClassType=initIO dataClassName=initIO unit='-' description='pneAux_TCV_pDmd_Rear_Right': IO_PNE_Generic.pneAux_TCV_pDmd_Rear_Right_0 [-]"; p667 "pneAux_trailerAxle1_left_stABSInValve (init) export=true name=pneAux_trailerAxle1_left_stABSInValve prio=1 dataSetName=std dataClassType=initIO dataClassName=initIO unit='-' description='pneAux_trailerAxle1_left_stABSInValve': IO_PNE_Generic.pneAux_trailerAxle1_left_stABSInValve_0 [-]"; p668 "pneAux_trailerAxle1_left_stABSOutValve (init) export=true name=pneAux_trailerAxle1_left_stABSOutValve prio=1 dataSetName=std dataClassType=initIO dataClassName=initIO unit='-' description='pneAux_trailerAxle1_left_stABSOutValve': IO_PNE_Generic.pneAux_trailerAxle1_left_stABSOutValve_0 [-]"; p669 "pneAux_trailerAxle1_load (init) export=true name=pneAux_trailerAxle1_load prio=1 dataSetName=std dataClassType=initIO dataClassName=initIO unit=kg description='pneAux_trailerAxle1_load': IO_PNE_Generic.pneAux_trailerAxle1_load_0 [-]"; p670 "pneAux_trailerAxle1_right_stABSInValve (init) export=true name=pneAux_trailerAxle1_right_stABSInValve prio=1 dataSetName=std dataClassType=initIO dataClassName=initIO unit='-' description='pneAux_trailerAxle1_right_stABSInValve': IO_PNE_Generic.pneAux_trailerAxle1_right_stABSInValve_0 [-]"; p671 "pneAux_trailerAxle1_right_stABSOutValve (init) export=true name=pneAux_trailerAxle1_right_stABSOutValve prio=1 dataSetName=std dataClassType=initIO dataClassName=initIO unit='-' description='pneAux_trailerAxle1_right_stABSOutValve': IO_PNE_Generic.pneAux_trailerAxle1_right_stABSOutValve_0 [-]"; p672 "pneAux_trailerAxle2_left_stABSInValve (init) export=true name=pneAux_trailerAxle2_left_stABSInValve prio=1 dataSetName=std dataClassType=initIO dataClassName=initIO unit='-' description='pneAux_trailerAxle2_left_stABSInValve': IO_PNE_Generic.pneAux_trailerAxle2_left_stABSInValve_0 [-]"; p673 "pneAux_trailerAxle2_left_stABSOutValve (init) export=true name=pneAux_trailerAxle2_left_stABSOutValve prio=1 dataSetName=std dataClassType=initIO dataClassName=initIO unit='-' description='pneAux_trailerAxle2_left_stABSOutValve': IO_PNE_Generic.pneAux_trailerAxle2_left_stABSOutValve_0 [-]"; p674 "pneAux_trailerAxle2_load (init) export=true name=pneAux_trailerAxle2_load prio=1 dataSetName=std dataClassType=initIO dataClassName=initIO unit=kg description='pneAux_trailerAxle2_load': IO_PNE_Generic.pneAux_trailerAxle2_load_0 [-]"; p675 "pneAux_trailerAxle2_right_stABSInValve (init) export=true name=pneAux_trailerAxle2_right_stABSInValve prio=1 dataSetName=std dataClassType=initIO dataClassName=initIO unit='-' description='pneAux_trailerAxle2_right_stABSInValve': IO_PNE_Generic.pneAux_trailerAxle2_right_stABSInValve_0 [-]"; p676 "pneAux_trailerAxle2_right_stABSOutValve (init) export=true name=pneAux_trailerAxle2_right_stABSOutValve prio=1 dataSetName=std dataClassType=initIO dataClassName=initIO unit='-' description='pneAux_trailerAxle2_right_stABSOutValve': IO_PNE_Generic.pneAux_trailerAxle2_right_stABSOutValve_0 [-]"; p677 "pneAux_trailerAxle3_left_stABSInValve (init) export=true name=pneAux_trailerAxle3_left_stABSInValve prio=1 dataSetName=std dataClassType=initIO dataClassName=initIO unit='-' description='pneAux_trailerAxle3_left_stABSInValve': IO_PNE_Generic.pneAux_trailerAxle3_left_stABSInValve_0 [-]"; p678 "pneAux_trailerAxle3_left_stABSOutValve (init) export=true name=pneAux_trailerAxle3_left_stABSOutValve prio=1 dataSetName=std dataClassType=initIO dataClassName=initIO unit='-' description='pneAux_trailerAxle3_left_stABSOutValve': IO_PNE_Generic.pneAux_trailerAxle3_left_stABSOutValve_0 [-]"; p679 "pneAux_trailerAxle3_load (init) export=true name=pneAux_trailerAxle3_load prio=1 dataSetName=std dataClassType=initIO dataClassName=initIO unit=kg description='pneAux_trailerAxle3_load': IO_PNE_Generic.pneAux_trailerAxle3_load_0 [-]"; p680 "pneAux_trailerAxle3_right_stABSInValve (init) export=true name=pneAux_trailerAxle3_right_stABSInValve prio=1 dataSetName=std dataClassType=initIO dataClassName=initIO unit='-' description='pneAux_trailerAxle3_right_stABSInValve': IO_PNE_Generic.pneAux_trailerAxle3_right_stABSInValve_0 [-]"; p681 "pneAux_trailerAxle3_right_stABSOutValve (init) export=true name=pneAux_trailerAxle3_right_stABSOutValve prio=1 dataSetName=std dataClassType=initIO dataClassName=initIO unit='-' description='pneAux_trailerAxle3_right_stABSOutValve': IO_PNE_Generic.pneAux_trailerAxle3_right_stABSOutValve_0 [-]"; p682 "Leakage Nominal Flow [l/min] export=true name=QnLeak prio=1 dataSetName=auxil_dummy dataClassType=auxil dataClassName=auxil unit='l' description='Leakage Nominal Flow [l/min]': leakageQn.QnLeak [-]"; p683 "step Size [s] export=true name=stepSize prio=1 dataSetName=veh_dummy dataClassType=veh dataClassName=veh unit='s' description=' step size [s]': pne3d_veh_Param.stepSize [s]"; p684 "Time Constant for Outlet Pressure Build Up APCV export=true name=T1_APCV prio=1 dataSetName=veh_dummy dataClassType=veh dataClassName=veh unit=s description='Time Constant for Outlet Pressure Build Up APCV': pne3d_veh_Param.T1_APCV [s]"; p685 "Time Constant for Outlet Pressure Build Up CMAX export=true name=T1_CMAX prio=1 dataSetName=veh_dummy dataClassType=veh dataClassName=veh unit=s description='Time Constant for Outlet Pressure Build Up CMAX': pne3d_veh_Param.T1_CMAX [s]"; p686 "Compressor Inlet Temperature Offset [K] export=true name=dT_CompInlet prio=1 dataSetName=pro_dummy dataClassType=pro dataClassName=pro unit='K' description='Compressor Inlet Temperature Offset [K]': pneumaticsParam.dT_CompInlet [-]"; p687 "US System Layout [0-false, 1-true,2-US6s6m] export=true name=flagUS prio=1 dataSetName=pro_dummy dataClassType=pro dataClassName=pro unit='-' description='US System Layout [0-false, 1-true,2-US6s6m]': pneumaticsParam.flagUS [-]"; p688 "Compressor Cut In Pressure (relative) at normal drive conditions [bar] export=true name=pRelCI prio=1 dataSetName=pro_dummy dataClassType=pro dataClassName=pro unit='bar' description='Compressor Cut In Pressure (relative) at normal drive conditions [bar]': pneumaticsParam.pRelCI [-]"; p689 "Compressor Cut In Pressure (relative) during Engine Run Over [bar] export=true name=pRelCI_RO prio=1 dataSetName=pro_dummy dataClassType=pro dataClassName=pro unit='bar' description='Compressor Cut In Pressure (relative) during Engine Run Over [bar]': pneumaticsParam.pRelCI_RO [-]"; p690 "Compressor Cut Off Pressure (relative) at normal drive conditions [bar] export=true name=pRelCO prio=1 dataSetName=pro_dummy dataClassType=pro dataClassName=pro unit='bar' description='Compressor Cut Off Pressure (relative) at normal drive conditions [bar]': pneumaticsParam.pRelCO [-]"; p691 "Compressor Cut Off Pressure (relative) during Engine Run Over [bar] export=true name=pRelCO_RO prio=1 dataSetName=pro_dummy dataClassType=pro dataClassName=pro unit='bar' description='Compressor Cut Off Pressure (relative) during Engine Run Over [bar]': pneumaticsParam.pRelCO_RO [-]"; p692 "EAPU Limitng Pressure (relative) primary circuits (V1, V2) [bar] export=true name=pRelLimit_C1C2 prio=1 dataSetName=pro_dummy dataClassType=pro dataClassName=pro unit='bar' description='EAPU Limitng Pressure (relative) primary circuits (V1, V2) [bar]': pneumaticsParam.pRelLimit_C1C2 [-]"; p693 "EAPU Limitng Pressure (relative) secondary circuits (V3, V4, V5, V6) [bar] export=true name=pRelLimit_C3C4 prio=1 dataSetName=pro_dummy dataClassType=pro dataClassName=pro unit='bar' description='EAPU Limitng Pressure (relative) secondary circuits (V3, V4, V5, V6) [bar]': pneumaticsParam.pRelLimit_C3C4 [-]"; p694 "EAPU Percentage of Regeneration [%] export=true name=RegenPct prio=1 dataSetName=pro_dummy dataClassType=pro dataClassName=pro unit='%' description='EAPU Percentage of Regeneration [%]': pneumaticsParam.RegenPct [-]"; p695 "Volume Tank1 [dm^3] export=true name=V1 prio=1 dataSetName=pro_dummy dataClassType=pro dataClassName=pro unit='dm^3' description='Volume Tank1 [dm^3]': pneumaticsParam.V1 [-]"; p696 "Volume Tank2 [dm^3] export=true name=V2 prio=1 dataSetName=pro_dummy dataClassType=pro dataClassName=pro unit='dm^3' description='Volume Tank2 [dm^3]': pneumaticsParam.V2 [-]"; p697 "Volume Tank3 [dm^3] export=true name=V3 prio=1 dataSetName=pro_dummy dataClassType=pro dataClassName=pro unit='dm^3' description='Volume Tank3 [dm^3]': pneumaticsParam.V3 [-]"; p698 "Volume Tank4 [dm^3] export=true name=V4 prio=1 dataSetName=pro_dummy dataClassType=pro dataClassName=pro unit='dm^3' description='Volume Tank4 [dm^3]': pneumaticsParam.V4 [-]"; p699 "Volume Tank5 [dm^3] export=true name=V5 prio=1 dataSetName=pro_dummy dataClassType=pro dataClassName=pro unit='dm^3' description='Volume Tank5 [dm^3]': pneumaticsParam.V5 [-]"; p700 "Volume Tank6 [dm^3] export=true name=V6 prio=1 dataSetName=pro_dummy dataClassType=pro dataClassName=pro unit='dm^3' description='Volume Tank6 [dm^3]': pneumaticsParam.V6 [-]"; p701 "Volume Tank7 [dm^3] export=true name=V7 prio=1 dataSetName=pro_dummy dataClassType=pro dataClassName=pro unit='dm^3' description='Volume Tank7 [dm^3]': pneumaticsParam.V7 [-]"; p702 "Volume Tank8 [dm^3] export=true name=V8 prio=1 dataSetName=pro_dummy dataClassType=pro dataClassName=pro unit='dm^3' description='Volume Tank8 [dm^3]': pneumaticsParam.V8 [-]"; p703 "Intake Volume of Cartridge [dm^3] export=true name=Vcartridge prio=1 dataSetName=pro_dummy dataClassType=pro dataClassName=pro unit='dm^3' description='Intake Volume of Cartridge [dm^3]': pneumaticsParam.Vcartridge [-]"; p704 "Intake Volume of Cooling Pipe [dm^3] export=true name=Vintake prio=1 dataSetName=pro_dummy dataClassType=pro dataClassName=pro unit='dm^3' description='Intake Volume of Cooling Pipe [dm^3]': pneumaticsParam.Vintake [-]"; p705 "Volume Tank Regeneration [dm^3] export=true name=Vreg prio=1 dataSetName=pro_dummy dataClassType=pro dataClassName=pro unit='dm^3' description='Volume Tank Regeneration [dm^3]': pneumaticsParam.Vreg [-]"; p706 "Volume Tank Supply [dm^3] export=true name=Vsup prio=1 dataSetName=pro_dummy dataClassType=pro dataClassName=pro unit='dm^3' description='Volume Tank Supply [dm^3]': pneumaticsParam.Vsup [-]"; p707 "SCR Nominal Flow [l/min] export=true name=QnSCR prio=1 dataSetName=auxil_dummy dataClassType=auxil dataClassName=auxil unit='l' description=SCR Nominal Flow [l/min]': SCR.QnSCR [-]"; p708 "temperatures calculation of brakes (0->No/1->Yes) export=true name=TemperatureCalculation prio=1 dataSetName=default dataClassType=initialTemperatures dataClassName=initialTemperatures unit='' description='temperatures calculation of brakes (0->No/1->Yes)': T_initial_brakes_Param.TemperatureCalculation [-]"; p709 "Air Consumption for Lifting of dxRef at Axle Load {mAxle, dV} [l] export=true name=dV_mAxle_Ref prio=1 dataSetName=susp_dummy dataClassType=susp dataClassName=$dataSetClassAirSpring$ unit='l' description='Air Consumption for Lifting of dxRef at Axle Load {mAxle, dV} [l]': airSpring_Axle1.dV_mAxle_Ref [-]"; p710 "Air Consumption for Lifting of dxRef at Axle Load {mAxle, dV} [l] export=true name=dV_mAxle_Ref prio=1 dataSetName=susp_dummy dataClassType=susp dataClassName=$dataSetClassAirSpring$ unit='l' description='Air Consumption for Lifting of dxRef at Axle Load {mAxle, dV} [l]': airSpring_Axle2.dV_mAxle_Ref [-]"; p711 "Air Consumption for Lifting of dxRef at Axle Load {mAxle, dV} [l] export=true name=dV_mAxle_Ref prio=1 dataSetName=susp_dummy dataClassType=susp dataClassName=$dataSetClassAirSpring$ unit='l' description='Air Consumption for Lifting of dxRef at Axle Load {mAxle, dV} [l]': airSpring_Axle3.dV_mAxle_Ref [-]"; p712 "Air Consumption for Lifting of dxRef at Axle Load {mAxle, dV} [l] export=true name=dV_mAxle_Ref prio=1 dataSetName=susp_dummy dataClassType=susp dataClassName=$dataSetClassAirSpring$ unit='l' description='Air Consumption for Lifting of dxRef at Axle Load {mAxle, dV} [l]': airSpring_Axle4.dV_mAxle_Ref [-]"; p713 "Temperature Values (x-Axis) of fac_T Temperature Correction Curve export=true name=fac_T_xAxis prio=1 dataSetName=brk_dummy dataClassType=brk dataClassName=$dataSetClassBrk$  unit='degC' description='Temperature Values in [degC] (x-Axis) of fac_T Temperature Correction Curve': BrakeA1_R.fac_T_xAxis [-]"; p714 "Correction Coefficient Values (y-Axis) of fac_T Temperature Correction Curve export=true name=fac_T_yAxis prio=1 dataSetName=brk_dummy dataClassType=brk dataClassName=$dataSetClassBrk$  unit='-' description='Correction Coefficient Values (y-Axis) of fac_T Temperature Correction Curve': BrakeA1_R.fac_T_yAxis [-]"; p715 "Velocity Values (x-Axis) of fac_v_Velocity Correction Curve export=true name=fac_v_xAxis prio=1 dataSetName=brk_dummy dataClassType=brk dataClassName=$dataSetClassBrk$  unit='m/s' description='Velocity Values (x-Axis) of fac_v_Velocity Correction Curve': BrakeA1_R.fac_v_xAxis [-]"; p716 "Correction Coefficient Values (y-Axis) of fac_v Temperature Correction Curve export=true name=fac_v_yAxis prio=1 dataSetName=brk_dummy dataClassType=brk dataClassName=$dataSetClassBrk$  unit='-' description='Correction Coefficient Values (y-Axis) of fac_v Velocity Correction Curve': BrakeA1_R.fac_v_yAxis [-]"; p717 "Force Values (x-Axis) of Lever Force-Displacement Curve export=true name=Fdx_xAxis prio=1 dataSetName=brk_dummy dataClassType=brk dataClassName=$dataSetClassBrk$  unit='N' description='Force Values (x-Axis) of Lever Force-Displacement Curve': BrakeA1_R.Fdx_xAxis [N]"; p718 "Displacement Values (y-Axis) of Lever Force-Displacement Curve export=true name=Fdx_yAxis prio=1 dataSetName=brk_dummy dataClassType=brk dataClassName=$dataSetClassBrk$  unit='m' description='Displacement Values (y-Axis) of Lever Force-Displacement Curve': BrakeA1_R.Fdx_yAxis [m]"; p719 "Displacement Values (x-Axis) of Lever Displacement-i Ratio Curve export=true name=i_xAxis prio=1 dataSetName=brk_dummy dataClassType=brk dataClassName=$dataSetClassBrk$  unit='m' description='Displacement Values (x-Axis) of Lever Displacement-i Ratio Curve': BrakeA1_R.i_xAxis [m]"; p720 "i Ratio Values (y-Axis) of Lever Displacement-i Ratio Curve export=true name=i_yAxis prio=1 dataSetName=brk_dummy dataClassType=brk dataClassName=$dataSetClassBrk$  unit='-' description='i Ratio Values (y-Axis) of Lever Displacement-i Ratio Curve': BrakeA1_R.i_yAxis [-]"; p721 "Temperature Values in [degC] (x-Axis) of wearRate-T-Curve export=true name=wearRate_T_xAxis prio=1 dataSetName=brk_dummy dataClassType=brk dataClassName=$dataSetClassBrk$  unit='degC' description='Temperature Values in [degC] (x-Axis) of wearRate-T-Curve': BrakeA1_R.wearRate_T_xAxis [-]"; p722 "Wear Rate Values (y-Axis) of wearRate-T-Curve [cm^3/kWh] export=true name=wearRate_T_yAxis prio=1 dataSetName=brk_dummy dataClassType=brk dataClassName=$dataSetClassBrk$  unit='-' description='Wear Rate Values (y-Axis) of wearRate-T-Curve [cm^3/kWh]': BrakeA1_R.wearRate_T_yAxis [-]"; p723 "Temperature Values (x-Axis) of fac_T Temperature Correction Curve export=true name=fac_T_xAxis prio=1 dataSetName=brk_dummy dataClassType=brk dataClassName=$dataSetClassBrk$  unit='degC' description='Temperature Values in [degC] (x-Axis) of fac_T Temperature Correction Curve': BrakeA2_R.fac_T_xAxis [-]"; p724 "Correction Coefficient Values (y-Axis) of fac_T Temperature Correction Curve export=true name=fac_T_yAxis prio=1 dataSetName=brk_dummy dataClassType=brk dataClassName=$dataSetClassBrk$  unit='-' description='Correction Coefficient Values (y-Axis) of fac_T Temperature Correction Curve': BrakeA2_R.fac_T_yAxis [-]"; p725 "Velocity Values (x-Axis) of fac_v_Velocity Correction Curve export=true name=fac_v_xAxis prio=1 dataSetName=brk_dummy dataClassType=brk dataClassName=$dataSetClassBrk$  unit='m/s' description='Velocity Values (x-Axis) of fac_v_Velocity Correction Curve': BrakeA2_R.fac_v_xAxis [-]"; p726 "Correction Coefficient Values (y-Axis) of fac_v Temperature Correction Curve export=true name=fac_v_yAxis prio=1 dataSetName=brk_dummy dataClassType=brk dataClassName=$dataSetClassBrk$  unit='-' description='Correction Coefficient Values (y-Axis) of fac_v Velocity Correction Curve': BrakeA2_R.fac_v_yAxis [-]"; p727 "Force Values (x-Axis) of Lever Force-Displacement Curve export=true name=Fdx_xAxis prio=1 dataSetName=brk_dummy dataClassType=brk dataClassName=$dataSetClassBrk$  unit='N' description='Force Values (x-Axis) of Lever Force-Displacement Curve': BrakeA2_R.Fdx_xAxis [N]"; p728 "Displacement Values (y-Axis) of Lever Force-Displacement Curve export=true name=Fdx_yAxis prio=1 dataSetName=brk_dummy dataClassType=brk dataClassName=$dataSetClassBrk$  unit='m' description='Displacement Values (y-Axis) of Lever Force-Displacement Curve': BrakeA2_R.Fdx_yAxis [m]"; p729 "Displacement Values (x-Axis) of Lever Displacement-i Ratio Curve export=true name=i_xAxis prio=1 dataSetName=brk_dummy dataClassType=brk dataClassName=$dataSetClassBrk$  unit='m' description='Displacement Values (x-Axis) of Lever Displacement-i Ratio Curve': BrakeA2_R.i_xAxis [m]"; p730 "i Ratio Values (y-Axis) of Lever Displacement-i Ratio Curve export=true name=i_yAxis prio=1 dataSetName=brk_dummy dataClassType=brk dataClassName=$dataSetClassBrk$  unit='-' description='i Ratio Values (y-Axis) of Lever Displacement-i Ratio Curve': BrakeA2_R.i_yAxis [-]"; p731 "Temperature Values in [degC] (x-Axis) of wearRate-T-Curve export=true name=wearRate_T_xAxis prio=1 dataSetName=brk_dummy dataClassType=brk dataClassName=$dataSetClassBrk$  unit='degC' description='Temperature Values in [degC] (x-Axis) of wearRate-T-Curve': BrakeA2_R.wearRate_T_xAxis [-]"; p732 "Wear Rate Values (y-Axis) of wearRate-T-Curve [cm^3/kWh] export=true name=wearRate_T_yAxis prio=1 dataSetName=brk_dummy dataClassType=brk dataClassName=$dataSetClassBrk$  unit='-' description='Wear Rate Values (y-Axis) of wearRate-T-Curve [cm^3/kWh]': BrakeA2_R.wearRate_T_yAxis [-]"; p733 "Temperature Values (x-Axis) of fac_T Temperature Correction Curve export=true name=fac_T_xAxis prio=1 dataSetName=brk_dummy dataClassType=brk dataClassName=$dataSetClassBrk$  unit='degC' description='Temperature Values in [degC] (x-Axis) of fac_T Temperature Correction Curve': BrakeA3_R.fac_T_xAxis [-]"; p734 "Correction Coefficient Values (y-Axis) of fac_T Temperature Correction Curve export=true name=fac_T_yAxis prio=1 dataSetName=brk_dummy dataClassType=brk dataClassName=$dataSetClassBrk$  unit='-' description='Correction Coefficient Values (y-Axis) of fac_T Temperature Correction Curve': BrakeA3_R.fac_T_yAxis [-]"; p735 "Velocity Values (x-Axis) of fac_v_Velocity Correction Curve export=true name=fac_v_xAxis prio=1 dataSetName=brk_dummy dataClassType=brk dataClassName=$dataSetClassBrk$  unit='m/s' description='Velocity Values (x-Axis) of fac_v_Velocity Correction Curve': BrakeA3_R.fac_v_xAxis [-]"; p736 "Correction Coefficient Values (y-Axis) of fac_v Temperature Correction Curve export=true name=fac_v_yAxis prio=1 dataSetName=brk_dummy dataClassType=brk dataClassName=$dataSetClassBrk$  unit='-' description='Correction Coefficient Values (y-Axis) of fac_v Velocity Correction Curve': BrakeA3_R.fac_v_yAxis [-]"; p737 "Force Values (x-Axis) of Lever Force-Displacement Curve export=true name=Fdx_xAxis prio=1 dataSetName=brk_dummy dataClassType=brk dataClassName=$dataSetClassBrk$  unit='N' description='Force Values (x-Axis) of Lever Force-Displacement Curve': BrakeA3_R.Fdx_xAxis [N]"; p738 "Displacement Values (y-Axis) of Lever Force-Displacement Curve export=true name=Fdx_yAxis prio=1 dataSetName=brk_dummy dataClassType=brk dataClassName=$dataSetClassBrk$  unit='m' description='Displacement Values (y-Axis) of Lever Force-Displacement Curve': BrakeA3_R.Fdx_yAxis [m]"; p739 "Displacement Values (x-Axis) of Lever Displacement-i Ratio Curve export=true name=i_xAxis prio=1 dataSetName=brk_dummy dataClassType=brk dataClassName=$dataSetClassBrk$  unit='m' description='Displacement Values (x-Axis) of Lever Displacement-i Ratio Curve': BrakeA3_R.i_xAxis [m]"; p740 "i Ratio Values (y-Axis) of Lever Displacement-i Ratio Curve export=true name=i_yAxis prio=1 dataSetName=brk_dummy dataClassType=brk dataClassName=$dataSetClassBrk$  unit='-' description='i Ratio Values (y-Axis) of Lever Displacement-i Ratio Curve': BrakeA3_R.i_yAxis [-]"; p741 "Temperature Values in [degC] (x-Axis) of wearRate-T-Curve export=true name=wearRate_T_xAxis prio=1 dataSetName=brk_dummy dataClassType=brk dataClassName=$dataSetClassBrk$  unit='degC' description='Temperature Values in [degC] (x-Axis) of wearRate-T-Curve': BrakeA3_R.wearRate_T_xAxis [-]"; p742 "Wear Rate Values (y-Axis) of wearRate-T-Curve [cm^3/kWh] export=true name=wearRate_T_yAxis prio=1 dataSetName=brk_dummy dataClassType=brk dataClassName=$dataSetClassBrk$  unit='-' description='Wear Rate Values (y-Axis) of wearRate-T-Curve [cm^3/kWh]': BrakeA3_R.wearRate_T_yAxis [-]"; p743 "Temperature Values (x-Axis) of fac_T Temperature Correction Curve export=true name=fac_T_xAxis prio=1 dataSetName=brk_dummy dataClassType=brk dataClassName=$dataSetClassBrk$  unit='degC' description='Temperature Values in [degC] (x-Axis) of fac_T Temperature Correction Curve': BrakeA4_R.fac_T_xAxis [-]"; p744 "Correction Coefficient Values (y-Axis) of fac_T Temperature Correction Curve export=true name=fac_T_yAxis prio=1 dataSetName=brk_dummy dataClassType=brk dataClassName=$dataSetClassBrk$  unit='-' description='Correction Coefficient Values (y-Axis) of fac_T Temperature Correction Curve': BrakeA4_R.fac_T_yAxis [-]"; p745 "Velocity Values (x-Axis) of fac_v_Velocity Correction Curve export=true name=fac_v_xAxis prio=1 dataSetName=brk_dummy dataClassType=brk dataClassName=$dataSetClassBrk$  unit='m/s' description='Velocity Values (x-Axis) of fac_v_Velocity Correction Curve': BrakeA4_R.fac_v_xAxis [-]"; p746 "Correction Coefficient Values (y-Axis) of fac_v Temperature Correction Curve export=true name=fac_v_yAxis prio=1 dataSetName=brk_dummy dataClassType=brk dataClassName=$dataSetClassBrk$  unit='-' description='Correction Coefficient Values (y-Axis) of fac_v Velocity Correction Curve': BrakeA4_R.fac_v_yAxis [-]"; p747 "Force Values (x-Axis) of Lever Force-Displacement Curve export=true name=Fdx_xAxis prio=1 dataSetName=brk_dummy dataClassType=brk dataClassName=$dataSetClassBrk$  unit='N' description='Force Values (x-Axis) of Lever Force-Displacement Curve': BrakeA4_R.Fdx_xAxis [N]"; p748 "Displacement Values (y-Axis) of Lever Force-Displacement Curve export=true name=Fdx_yAxis prio=1 dataSetName=brk_dummy dataClassType=brk dataClassName=$dataSetClassBrk$  unit='m' description='Displacement Values (y-Axis) of Lever Force-Displacement Curve': BrakeA4_R.Fdx_yAxis [m]"; p749 "Displacement Values (x-Axis) of Lever Displacement-i Ratio Curve export=true name=i_xAxis prio=1 dataSetName=brk_dummy dataClassType=brk dataClassName=$dataSetClassBrk$  unit='m' description='Displacement Values (x-Axis) of Lever Displacement-i Ratio Curve': BrakeA4_R.i_xAxis [m]"; p750 "i Ratio Values (y-Axis) of Lever Displacement-i Ratio Curve export=true name=i_yAxis prio=1 dataSetName=brk_dummy dataClassType=brk dataClassName=$dataSetClassBrk$  unit='-' description='i Ratio Values (y-Axis) of Lever Displacement-i Ratio Curve': BrakeA4_R.i_yAxis [-]"; p751 "Temperature Values in [degC] (x-Axis) of wearRate-T-Curve export=true name=wearRate_T_xAxis prio=1 dataSetName=brk_dummy dataClassType=brk dataClassName=$dataSetClassBrk$  unit='degC' description='Temperature Values in [degC] (x-Axis) of wearRate-T-Curve': BrakeA4_R.wearRate_T_xAxis [-]"; p752 "Wear Rate Values (y-Axis) of wearRate-T-Curve [cm^3/kWh] export=true name=wearRate_T_yAxis prio=1 dataSetName=brk_dummy dataClassType=brk dataClassName=$dataSetClassBrk$  unit='-' description='Wear Rate Values (y-Axis) of wearRate-T-Curve [cm^3/kWh]': BrakeA4_R.wearRate_T_yAxis [-]"; p753 "dx Values (x-axis) for dx-Spring Brake Force Curve export=true name=dxFSpring_xAxis prio=1 dataSetName=cyl_dummy dataClassType=cyl dataClassName=$dataSetClassCyl$  unit='m' description='dx Values (x-axis) for dx-Spring Brake Force Curve': brakeCylinderA1_R.dxFSpring_xAxis [m]"; p754 "Force Values (y-axis) for dx-Spring Brake Force Curve export=true name=dxFSpring_yAxis prio=1 dataSetName=cyl_dummy dataClassType=cyl dataClassName=$dataSetClassCyl$  unit='N' description='Force Values (y-axis) for dx-Spring Brake Force Curve': brakeCylinderA1_R.dxFSpring_yAxis [N]"; p755 "dx Values (x-axis) for dx-Volume Intake Curve Parking Brake export=true name=dxVolPB_xAxis prio=1 dataSetName=cyl_dummy dataClassType=cyl dataClassName=$dataSetClassCyl$  unit='m' description='dx Values (x-axis) for dx-Volume Intake Curve Parking Brake': brakeCylinderA1_R.dxVolPB_xAxis [m]"; p756 "Volume Values (y-axis) for dx-Volume Intake Curve Parking Brake export=true name=dxVolPB_yAxis prio=1 dataSetName=cyl_dummy dataClassType=cyl dataClassName=$dataSetClassCyl$  unit='m^3' description='Volume Values (y-axis) for dx-Volume Intake Curve Parking Brake': brakeCylinderA1_R.dxVolPB_yAxis [m³]"; p757 "dx Values (x-axis) for dx-Volume Intake Curve Service Brake export=true name=dxVolSB_xAxis prio=1 dataSetName=cyl_dummy dataClassType=cyl dataClassName=$dataSetClassCyl$  unit='m' description='dx Values (x-axis) for dx-Volume Intake Curve Service Brake': brakeCylinderA1_R.dxVolSB_xAxis [m]"; p758 "Volume Values (y-axis) for dx-Volume Intake Curve Service Brake export=true name=dxVolSB_yAxis prio=1 dataSetName=cyl_dummy dataClassType=cyl dataClassName=$dataSetClassCyl$  unit='m^3' description='Volume Values (y-axis) for dx-Volume Intake Curve Service Brake': brakeCylinderA1_R.dxVolSB_yAxis [m³]"; p759 "dx Values (x-axis) for dx-Spring Brake Force Curve export=true name=dxFSpring_xAxis prio=1 dataSetName=cyl_dummy dataClassType=cyl dataClassName=$dataSetClassCyl$  unit='m' description='dx Values (x-axis) for dx-Spring Brake Force Curve': brakeCylinderA2_R.dxFSpring_xAxis [m]"; p760 "Force Values (y-axis) for dx-Spring Brake Force Curve export=true name=dxFSpring_yAxis prio=1 dataSetName=cyl_dummy dataClassType=cyl dataClassName=$dataSetClassCyl$  unit='N' description='Force Values (y-axis) for dx-Spring Brake Force Curve': brakeCylinderA2_R.dxFSpring_yAxis [N]"; p761 "dx Values (x-axis) for dx-Volume Intake Curve Parking Brake export=true name=dxVolPB_xAxis prio=1 dataSetName=cyl_dummy dataClassType=cyl dataClassName=$dataSetClassCyl$  unit='m' description='dx Values (x-axis) for dx-Volume Intake Curve Parking Brake': brakeCylinderA2_R.dxVolPB_xAxis [m]"; p762 "Volume Values (y-axis) for dx-Volume Intake Curve Parking Brake export=true name=dxVolPB_yAxis prio=1 dataSetName=cyl_dummy dataClassType=cyl dataClassName=$dataSetClassCyl$  unit='m^3' description='Volume Values (y-axis) for dx-Volume Intake Curve Parking Brake': brakeCylinderA2_R.dxVolPB_yAxis [m³]"; p763 "dx Values (x-axis) for dx-Volume Intake Curve Service Brake export=true name=dxVolSB_xAxis prio=1 dataSetName=cyl_dummy dataClassType=cyl dataClassName=$dataSetClassCyl$  unit='m' description='dx Values (x-axis) for dx-Volume Intake Curve Service Brake': brakeCylinderA2_R.dxVolSB_xAxis [m]"; p764 "Volume Values (y-axis) for dx-Volume Intake Curve Service Brake export=true name=dxVolSB_yAxis prio=1 dataSetName=cyl_dummy dataClassType=cyl dataClassName=$dataSetClassCyl$  unit='m^3' description='Volume Values (y-axis) for dx-Volume Intake Curve Service Brake': brakeCylinderA2_R.dxVolSB_yAxis [m³]"; p765 "dx Values (x-axis) for dx-Spring Brake Force Curve export=true name=dxFSpring_xAxis prio=1 dataSetName=cyl_dummy dataClassType=cyl dataClassName=$dataSetClassCyl$  unit='m' description='dx Values (x-axis) for dx-Spring Brake Force Curve': brakeCylinderA3_R.dxFSpring_xAxis [m]"; p766 "Force Values (y-axis) for dx-Spring Brake Force Curve export=true name=dxFSpring_yAxis prio=1 dataSetName=cyl_dummy dataClassType=cyl dataClassName=$dataSetClassCyl$  unit='N' description='Force Values (y-axis) for dx-Spring Brake Force Curve': brakeCylinderA3_R.dxFSpring_yAxis [N]"; p767 "dx Values (x-axis) for dx-Volume Intake Curve Parking Brake export=true name=dxVolPB_xAxis prio=1 dataSetName=cyl_dummy dataClassType=cyl dataClassName=$dataSetClassCyl$  unit='m' description='dx Values (x-axis) for dx-Volume Intake Curve Parking Brake': brakeCylinderA3_R.dxVolPB_xAxis [m]"; p768 "Volume Values (y-axis) for dx-Volume Intake Curve Parking Brake export=true name=dxVolPB_yAxis prio=1 dataSetName=cyl_dummy dataClassType=cyl dataClassName=$dataSetClassCyl$  unit='m^3' description='Volume Values (y-axis) for dx-Volume Intake Curve Parking Brake': brakeCylinderA3_R.dxVolPB_yAxis [m³]"; p769 "dx Values (x-axis) for dx-Volume Intake Curve Service Brake export=true name=dxVolSB_xAxis prio=1 dataSetName=cyl_dummy dataClassType=cyl dataClassName=$dataSetClassCyl$  unit='m' description='dx Values (x-axis) for dx-Volume Intake Curve Service Brake': brakeCylinderA3_R.dxVolSB_xAxis [m]"; p770 "Volume Values (y-axis) for dx-Volume Intake Curve Service Brake export=true name=dxVolSB_yAxis prio=1 dataSetName=cyl_dummy dataClassType=cyl dataClassName=$dataSetClassCyl$  unit='m^3' description='Volume Values (y-axis) for dx-Volume Intake Curve Service Brake': brakeCylinderA3_R.dxVolSB_yAxis [m³]"; p771 "dx Values (x-axis) for dx-Spring Brake Force Curve export=true name=dxFSpring_xAxis prio=1 dataSetName=cyl_dummy dataClassType=cyl dataClassName=$dataSetClassCyl$  unit='m' description='dx Values (x-axis) for dx-Spring Brake Force Curve': brakeCylinderA4_R.dxFSpring_xAxis [m]"; p772 "Force Values (y-axis) for dx-Spring Brake Force Curve export=true name=dxFSpring_yAxis prio=1 dataSetName=cyl_dummy dataClassType=cyl dataClassName=$dataSetClassCyl$  unit='N' description='Force Values (y-axis) for dx-Spring Brake Force Curve': brakeCylinderA4_R.dxFSpring_yAxis [N]"; p773 "dx Values (x-axis) for dx-Volume Intake Curve Parking Brake export=true name=dxVolPB_xAxis prio=1 dataSetName=cyl_dummy dataClassType=cyl dataClassName=$dataSetClassCyl$  unit='m' description='dx Values (x-axis) for dx-Volume Intake Curve Parking Brake': brakeCylinderA4_R.dxVolPB_xAxis [m]"; p774 "Volume Values (y-axis) for dx-Volume Intake Curve Parking Brake export=true name=dxVolPB_yAxis prio=1 dataSetName=cyl_dummy dataClassType=cyl dataClassName=$dataSetClassCyl$  unit='m^3' description='Volume Values (y-axis) for dx-Volume Intake Curve Parking Brake': brakeCylinderA4_R.dxVolPB_yAxis [m³]"; p775 "dx Values (x-axis) for dx-Volume Intake Curve Service Brake export=true name=dxVolSB_xAxis prio=1 dataSetName=cyl_dummy dataClassType=cyl dataClassName=$dataSetClassCyl$  unit='m' description='dx Values (x-axis) for dx-Volume Intake Curve Service Brake': brakeCylinderA4_R.dxVolSB_xAxis [m]"; p776 "Volume Values (y-axis) for dx-Volume Intake Curve Service Brake export=true name=dxVolSB_yAxis prio=1 dataSetName=cyl_dummy dataClassType=cyl dataClassName=$dataSetClassCyl$  unit='m^3' description='Volume Values (y-axis) for dx-Volume Intake Curve Service Brake': brakeCylinderA4_R.dxVolSB_yAxis [m³]"; p777 "dx Values (x-axis) for dx-Spring Brake Force Curve export=true name=dxFSpring_xAxis prio=1 dataSetName=cyl_dummy dataClassType=cyl dataClassName=$dataSetClassCyl$  unit='m' description='dx Values (x-axis) for dx-Spring Brake Force Curve': brakeCylinderTrailerA1_R.dxFSpring_xAxis [m]"; p778 "Force Values (y-axis) for dx-Spring Brake Force Curve export=true name=dxFSpring_yAxis prio=1 dataSetName=cyl_dummy dataClassType=cyl dataClassName=$dataSetClassCyl$  unit='N' description='Force Values (y-axis) for dx-Spring Brake Force Curve': brakeCylinderTrailerA1_R.dxFSpring_yAxis [N]"; p779 "dx Values (x-axis) for dx-Volume Intake Curve Parking Brake export=true name=dxVolPB_xAxis prio=1 dataSetName=cyl_dummy dataClassType=cyl dataClassName=$dataSetClassCyl$  unit='m' description='dx Values (x-axis) for dx-Volume Intake Curve Parking Brake': brakeCylinderTrailerA1_R.dxVolPB_xAxis [m]"; p780 "Volume Values (y-axis) for dx-Volume Intake Curve Parking Brake export=true name=dxVolPB_yAxis prio=1 dataSetName=cyl_dummy dataClassType=cyl dataClassName=$dataSetClassCyl$  unit='m^3' description='Volume Values (y-axis) for dx-Volume Intake Curve Parking Brake': brakeCylinderTrailerA1_R.dxVolPB_yAxis [m³]"; p781 "dx Values (x-axis) for dx-Volume Intake Curve Service Brake export=true name=dxVolSB_xAxis prio=1 dataSetName=cyl_dummy dataClassType=cyl dataClassName=$dataSetClassCyl$  unit='m' description='dx Values (x-axis) for dx-Volume Intake Curve Service Brake': brakeCylinderTrailerA1_R.dxVolSB_xAxis [m]"; p782 "Volume Values (y-axis) for dx-Volume Intake Curve Service Brake export=true name=dxVolSB_yAxis prio=1 dataSetName=cyl_dummy dataClassType=cyl dataClassName=$dataSetClassCyl$  unit='m^3' description='Volume Values (y-axis) for dx-Volume Intake Curve Service Brake': brakeCylinderTrailerA1_R.dxVolSB_yAxis [m³]"; p783 "dx Values (x-axis) for dx-Spring Brake Force Curve export=true name=dxFSpring_xAxis prio=1 dataSetName=cyl_dummy dataClassType=cyl dataClassName=$dataSetClassCyl$  unit='m' description='dx Values (x-axis) for dx-Spring Brake Force Curve': brakeCylinderTrailerA2_R.dxFSpring_xAxis [m]"; p784 "Force Values (y-axis) for dx-Spring Brake Force Curve export=true name=dxFSpring_yAxis prio=1 dataSetName=cyl_dummy dataClassType=cyl dataClassName=$dataSetClassCyl$  unit='N' description='Force Values (y-axis) for dx-Spring Brake Force Curve': brakeCylinderTrailerA2_R.dxFSpring_yAxis [N]"; p785 "dx Values (x-axis) for dx-Volume Intake Curve Parking Brake export=true name=dxVolPB_xAxis prio=1 dataSetName=cyl_dummy dataClassType=cyl dataClassName=$dataSetClassCyl$  unit='m' description='dx Values (x-axis) for dx-Volume Intake Curve Parking Brake': brakeCylinderTrailerA2_R.dxVolPB_xAxis [m]"; p786 "Volume Values (y-axis) for dx-Volume Intake Curve Parking Brake export=true name=dxVolPB_yAxis prio=1 dataSetName=cyl_dummy dataClassType=cyl dataClassName=$dataSetClassCyl$  unit='m^3' description='Volume Values (y-axis) for dx-Volume Intake Curve Parking Brake': brakeCylinderTrailerA2_R.dxVolPB_yAxis [m³]"; p787 "dx Values (x-axis) for dx-Volume Intake Curve Service Brake export=true name=dxVolSB_xAxis prio=1 dataSetName=cyl_dummy dataClassType=cyl dataClassName=$dataSetClassCyl$  unit='m' description='dx Values (x-axis) for dx-Volume Intake Curve Service Brake': brakeCylinderTrailerA2_R.dxVolSB_xAxis [m]"; p788 "Volume Values (y-axis) for dx-Volume Intake Curve Service Brake export=true name=dxVolSB_yAxis prio=1 dataSetName=cyl_dummy dataClassType=cyl dataClassName=$dataSetClassCyl$  unit='m^3' description='Volume Values (y-axis) for dx-Volume Intake Curve Service Brake': brakeCylinderTrailerA2_R.dxVolSB_yAxis [m³]"; p789 "dx Values (x-axis) for dx-Spring Brake Force Curve export=true name=dxFSpring_xAxis prio=1 dataSetName=cyl_dummy dataClassType=cyl dataClassName=$dataSetClassCyl$  unit='m' description='dx Values (x-axis) for dx-Spring Brake Force Curve': brakeCylinderTrailerA3_R.dxFSpring_xAxis [m]"; p790 "Force Values (y-axis) for dx-Spring Brake Force Curve export=true name=dxFSpring_yAxis prio=1 dataSetName=cyl_dummy dataClassType=cyl dataClassName=$dataSetClassCyl$  unit='N' description='Force Values (y-axis) for dx-Spring Brake Force Curve': brakeCylinderTrailerA3_R.dxFSpring_yAxis [N]"; p791 "dx Values (x-axis) for dx-Volume Intake Curve Parking Brake export=true name=dxVolPB_xAxis prio=1 dataSetName=cyl_dummy dataClassType=cyl dataClassName=$dataSetClassCyl$  unit='m' description='dx Values (x-axis) for dx-Volume Intake Curve Parking Brake': brakeCylinderTrailerA3_R.dxVolPB_xAxis [m]"; p792 "Volume Values (y-axis) for dx-Volume Intake Curve Parking Brake export=true name=dxVolPB_yAxis prio=1 dataSetName=cyl_dummy dataClassType=cyl dataClassName=$dataSetClassCyl$  unit='m^3' description='Volume Values (y-axis) for dx-Volume Intake Curve Parking Brake': brakeCylinderTrailerA3_R.dxVolPB_yAxis [m³]"; p793 "dx Values (x-axis) for dx-Volume Intake Curve Service Brake export=true name=dxVolSB_xAxis prio=1 dataSetName=cyl_dummy dataClassType=cyl dataClassName=$dataSetClassCyl$  unit='m' description='dx Values (x-axis) for dx-Volume Intake Curve Service Brake': brakeCylinderTrailerA3_R.dxVolSB_xAxis [m]"; p794 "Volume Values (y-axis) for dx-Volume Intake Curve Service Brake export=true name=dxVolSB_yAxis prio=1 dataSetName=cyl_dummy dataClassType=cyl dataClassName=$dataSetClassCyl$  unit='m^3' description='Volume Values (y-axis) for dx-Volume Intake Curve Service Brake': brakeCylinderTrailerA3_R.dxVolSB_yAxis [m³]"; p795 "Temperature Values (x-Axis) of fac_T Temperature Correction Curve export=true name=fac_T_xAxis prio=1 dataSetName=brk_dummy dataClassType=brk dataClassName=$dataSetClassBrk$  unit='degC' description='Temperature Values in [degC] (x-Axis) of fac_T Temperature Correction Curve': BrakeTrailerA1_R.fac_T_xAxis [-]"; p796 "Correction Coefficient Values (y-Axis) of fac_T Temperature Correction Curve export=true name=fac_T_yAxis prio=1 dataSetName=brk_dummy dataClassType=brk dataClassName=$dataSetClassBrk$  unit='-' description='Correction Coefficient Values (y-Axis) of fac_T Temperature Correction Curve': BrakeTrailerA1_R.fac_T_yAxis [-]"; p797 "Velocity Values (x-Axis) of fac_v_Velocity Correction Curve export=true name=fac_v_xAxis prio=1 dataSetName=brk_dummy dataClassType=brk dataClassName=$dataSetClassBrk$  unit='m/s' description='Velocity Values (x-Axis) of fac_v_Velocity Correction Curve': BrakeTrailerA1_R.fac_v_xAxis [-]"; p798 "Correction Coefficient Values (y-Axis) of fac_v Temperature Correction Curve export=true name=fac_v_yAxis prio=1 dataSetName=brk_dummy dataClassType=brk dataClassName=$dataSetClassBrk$  unit='-' description='Correction Coefficient Values (y-Axis) of fac_v Velocity Correction Curve': BrakeTrailerA1_R.fac_v_yAxis [-]"; p799 "Force Values (x-Axis) of Lever Force-Displacement Curve export=true name=Fdx_xAxis prio=1 dataSetName=brk_dummy dataClassType=brk dataClassName=$dataSetClassBrk$  unit='N' description='Force Values (x-Axis) of Lever Force-Displacement Curve': BrakeTrailerA1_R.Fdx_xAxis [N]"; p800 "Displacement Values (y-Axis) of Lever Force-Displacement Curve export=true name=Fdx_yAxis prio=1 dataSetName=brk_dummy dataClassType=brk dataClassName=$dataSetClassBrk$  unit='m' description='Displacement Values (y-Axis) of Lever Force-Displacement Curve': BrakeTrailerA1_R.Fdx_yAxis [m]"; p801 "Displacement Values (x-Axis) of Lever Displacement-i Ratio Curve export=true name=i_xAxis prio=1 dataSetName=brk_dummy dataClassType=brk dataClassName=$dataSetClassBrk$  unit='m' description='Displacement Values (x-Axis) of Lever Displacement-i Ratio Curve': BrakeTrailerA1_R.i_xAxis [m]"; p802 "i Ratio Values (y-Axis) of Lever Displacement-i Ratio Curve export=true name=i_yAxis prio=1 dataSetName=brk_dummy dataClassType=brk dataClassName=$dataSetClassBrk$  unit='-' description='i Ratio Values (y-Axis) of Lever Displacement-i Ratio Curve': BrakeTrailerA1_R.i_yAxis [-]"; p803 "Temperature Values in [degC] (x-Axis) of wearRate-T-Curve export=true name=wearRate_T_xAxis prio=1 dataSetName=brk_dummy dataClassType=brk dataClassName=$dataSetClassBrk$  unit='degC' description='Temperature Values in [degC] (x-Axis) of wearRate-T-Curve': BrakeTrailerA1_R.wearRate_T_xAxis [-]"; p804 "Wear Rate Values (y-Axis) of wearRate-T-Curve [cm^3/kWh] export=true name=wearRate_T_yAxis prio=1 dataSetName=brk_dummy dataClassType=brk dataClassName=$dataSetClassBrk$  unit='-' description='Wear Rate Values (y-Axis) of wearRate-T-Curve [cm^3/kWh]': BrakeTrailerA1_R.wearRate_T_yAxis [-]"; p805 "Temperature Values (x-Axis) of fac_T Temperature Correction Curve export=true name=fac_T_xAxis prio=1 dataSetName=brk_dummy dataClassType=brk dataClassName=$dataSetClassBrk$  unit='degC' description='Temperature Values in [degC] (x-Axis) of fac_T Temperature Correction Curve': BrakeTrailerA2_R.fac_T_xAxis [-]"; p806 "Correction Coefficient Values (y-Axis) of fac_T Temperature Correction Curve export=true name=fac_T_yAxis prio=1 dataSetName=brk_dummy dataClassType=brk dataClassName=$dataSetClassBrk$  unit='-' description='Correction Coefficient Values (y-Axis) of fac_T Temperature Correction Curve': BrakeTrailerA2_R.fac_T_yAxis [-]"; p807 "Velocity Values (x-Axis) of fac_v_Velocity Correction Curve export=true name=fac_v_xAxis prio=1 dataSetName=brk_dummy dataClassType=brk dataClassName=$dataSetClassBrk$  unit='m/s' description='Velocity Values (x-Axis) of fac_v_Velocity Correction Curve': BrakeTrailerA2_R.fac_v_xAxis [-]"; p808 "Correction Coefficient Values (y-Axis) of fac_v Temperature Correction Curve export=true name=fac_v_yAxis prio=1 dataSetName=brk_dummy dataClassType=brk dataClassName=$dataSetClassBrk$  unit='-' description='Correction Coefficient Values (y-Axis) of fac_v Velocity Correction Curve': BrakeTrailerA2_R.fac_v_yAxis [-]"; p809 "Force Values (x-Axis) of Lever Force-Displacement Curve export=true name=Fdx_xAxis prio=1 dataSetName=brk_dummy dataClassType=brk dataClassName=$dataSetClassBrk$  unit='N' description='Force Values (x-Axis) of Lever Force-Displacement Curve': BrakeTrailerA2_R.Fdx_xAxis [N]"; p810 "Displacement Values (y-Axis) of Lever Force-Displacement Curve export=true name=Fdx_yAxis prio=1 dataSetName=brk_dummy dataClassType=brk dataClassName=$dataSetClassBrk$  unit='m' description='Displacement Values (y-Axis) of Lever Force-Displacement Curve': BrakeTrailerA2_R.Fdx_yAxis [m]"; p811 "Displacement Values (x-Axis) of Lever Displacement-i Ratio Curve export=true name=i_xAxis prio=1 dataSetName=brk_dummy dataClassType=brk dataClassName=$dataSetClassBrk$  unit='m' description='Displacement Values (x-Axis) of Lever Displacement-i Ratio Curve': BrakeTrailerA2_R.i_xAxis [m]"; p812 "i Ratio Values (y-Axis) of Lever Displacement-i Ratio Curve export=true name=i_yAxis prio=1 dataSetName=brk_dummy dataClassType=brk dataClassName=$dataSetClassBrk$  unit='-' description='i Ratio Values (y-Axis) of Lever Displacement-i Ratio Curve': BrakeTrailerA2_R.i_yAxis [-]"; p813 "Temperature Values in [degC] (x-Axis) of wearRate-T-Curve export=true name=wearRate_T_xAxis prio=1 dataSetName=brk_dummy dataClassType=brk dataClassName=$dataSetClassBrk$  unit='degC' description='Temperature Values in [degC] (x-Axis) of wearRate-T-Curve': BrakeTrailerA2_R.wearRate_T_xAxis [-]"; p814 "Wear Rate Values (y-Axis) of wearRate-T-Curve [cm^3/kWh] export=true name=wearRate_T_yAxis prio=1 dataSetName=brk_dummy dataClassType=brk dataClassName=$dataSetClassBrk$  unit='-' description='Wear Rate Values (y-Axis) of wearRate-T-Curve [cm^3/kWh]': BrakeTrailerA2_R.wearRate_T_yAxis [-]"; p815 "Temperature Values (x-Axis) of fac_T Temperature Correction Curve export=true name=fac_T_xAxis prio=1 dataSetName=brk_dummy dataClassType=brk dataClassName=$dataSetClassBrk$  unit='degC' description='Temperature Values in [degC] (x-Axis) of fac_T Temperature Correction Curve': BrakeTrailerA3_R.fac_T_xAxis [-]"; p816 "Correction Coefficient Values (y-Axis) of fac_T Temperature Correction Curve export=true name=fac_T_yAxis prio=1 dataSetName=brk_dummy dataClassType=brk dataClassName=$dataSetClassBrk$  unit='-' description='Correction Coefficient Values (y-Axis) of fac_T Temperature Correction Curve': BrakeTrailerA3_R.fac_T_yAxis [-]"; p817 "Velocity Values (x-Axis) of fac_v_Velocity Correction Curve export=true name=fac_v_xAxis prio=1 dataSetName=brk_dummy dataClassType=brk dataClassName=$dataSetClassBrk$  unit='m/s' description='Velocity Values (x-Axis) of fac_v_Velocity Correction Curve': BrakeTrailerA3_R.fac_v_xAxis [-]"; p818 "Correction Coefficient Values (y-Axis) of fac_v Temperature Correction Curve export=true name=fac_v_yAxis prio=1 dataSetName=brk_dummy dataClassType=brk dataClassName=$dataSetClassBrk$  unit='-' description='Correction Coefficient Values (y-Axis) of fac_v Velocity Correction Curve': BrakeTrailerA3_R.fac_v_yAxis [-]"; p819 "Force Values (x-Axis) of Lever Force-Displacement Curve export=true name=Fdx_xAxis prio=1 dataSetName=brk_dummy dataClassType=brk dataClassName=$dataSetClassBrk$  unit='N' description='Force Values (x-Axis) of Lever Force-Displacement Curve': BrakeTrailerA3_R.Fdx_xAxis [N]"; p820 "Displacement Values (y-Axis) of Lever Force-Displacement Curve export=true name=Fdx_yAxis prio=1 dataSetName=brk_dummy dataClassType=brk dataClassName=$dataSetClassBrk$  unit='m' description='Displacement Values (y-Axis) of Lever Force-Displacement Curve': BrakeTrailerA3_R.Fdx_yAxis [m]"; p821 "Displacement Values (x-Axis) of Lever Displacement-i Ratio Curve export=true name=i_xAxis prio=1 dataSetName=brk_dummy dataClassType=brk dataClassName=$dataSetClassBrk$  unit='m' description='Displacement Values (x-Axis) of Lever Displacement-i Ratio Curve': BrakeTrailerA3_R.i_xAxis [m]"; p822 "i Ratio Values (y-Axis) of Lever Displacement-i Ratio Curve export=true name=i_yAxis prio=1 dataSetName=brk_dummy dataClassType=brk dataClassName=$dataSetClassBrk$  unit='-' description='i Ratio Values (y-Axis) of Lever Displacement-i Ratio Curve': BrakeTrailerA3_R.i_yAxis [-]"; p823 "Temperature Values in [degC] (x-Axis) of wearRate-T-Curve export=true name=wearRate_T_xAxis prio=1 dataSetName=brk_dummy dataClassType=brk dataClassName=$dataSetClassBrk$  unit='degC' description='Temperature Values in [degC] (x-Axis) of wearRate-T-Curve': BrakeTrailerA3_R.wearRate_T_xAxis [-]"; p824 "Wear Rate Values (y-Axis) of wearRate-T-Curve [cm^3/kWh] export=true name=wearRate_T_yAxis prio=1 dataSetName=brk_dummy dataClassType=brk dataClassName=$dataSetClassBrk$  unit='-' description='Wear Rate Values (y-Axis) of wearRate-T-Curve [cm^3/kWh]': BrakeTrailerA3_R.wearRate_T_yAxis [-]"; p825 "Brake Circuit Configuration [A1, A2, A3, A4] (0-Dummy, 1-Front, 2-Rear, 3-Middle(Bus)) export=true name=brkCircuit prio=1 dataSetName=circ_dummy dataClassType=circ dataClassName=circ unit='-' description='Brake Circuit Configuration [A1, A2, A3, A4] (0-Dummy, 1-Front, 2-Rear, 3-Middle(Bus))': brkCircuit.brkCircuit [-]"; p826 "Vehicle Speed Sensor Axle Position {A1,A2,A3,A4} (0-false,1-true)  export=true name=speedSensorPosnVeh prio=1 dataSetName=circ_dummy dataClassType=circ dataClassName=circ unit='' description='Vehicle Speed Sensor Axle Position {A1,A2,A3,A4} (0-false,1-true)': brkCircuit.speedSensorPosnVeh [-]"; p827 "Pressure Rise Time to 75% of asymptodic pressure value in [s] [A1, A2, A3, A4] export=true name=t_asymp75 prio=1 dataSetName=circ_dummy dataClassType=circ dataClassName=circ unit='-' description='Pressure Rise Time to 75% of asymptodic pressure value in [s] [A1, A2, A3, A4]': brkCircuit.t_asymp75 [-]"; p828 "Pressure Release Time from 100% to 10% of asymptodic pressure value in [s] [A1, A2, A3, A4] export=true name=t_release10 prio=1 dataSetName=circ_dummy dataClassType=circ dataClassName=circ unit='-' description='Pressure Release Time from 100% to 10% of asymptodic pressure value in [s] [A1, A2, A3, A4]': brkCircuit.t_release10 [-]"; p829 "Brake Circuit Configuration [TA1, TA2, TA3] (0-Dummy, 1-Front, 2-Rear) export=true name=brkCircuitTrailer prio=1 dataSetName=circTrlr_dummy dataClassType=circTrlr dataClassName=circTrlr unit='-' description='Brake Circuit Configuration Trailer [TA1, TA2, TA3] (0-Dummy, 1-Front, 2-Rear)': brkCircuitTrlr.brkCircuitTrailer [-]"; p830 "Trailer Control Active / Trailer can brake (0 - no, 1- yes ALB lower limit, 2- yes ALB normal, 3- yes ALB upper limit , 4 - yes without ALB) export=true name=flagTrailerControlActive prio=1 dataSetName=circTrlr_dummy dataClassType=circTrlr dataClassName=circTrlr unit='-' description='Trailer Control Active / Trailer can brake (0 - no, 1- yes ALB lower limit, 2- yes ALB normal, 3- yes ALB upper limit , 4 - yes without ALB)': brkCircuitTrlr.flagTrailerControlActive [-]"; p831 "Trailer Speed Sensor Axle Position [0-false,1-true] {A1,A2,A3}, used in pneAux export=true name=speedSensorPosnTrailer prio=1 dataSetName=circTrlr_dummy dataClassType=circTrlr dataClassName=circTrlr unit='-' description='Trailer Speed Sensor Axle Position [0-false,1-true] {A1,A2,A3}': brkCircuitTrlr.speedSensorPosnTrailer [-]"; p832 "Pressure Rise Time to 75% of asymptodic pressure value in [s] [TA1, TA2, TA3] export=true name=t_asymp75_Trlr prio=1 dataSetName=circTrlr_dummy dataClassType=circTrlr dataClassName=circTrlr unit='-' description='Pressure Rise Time to 75% of asymptodic pressure value in [s] [TA1, TA2, TA3]': brkCircuitTrlr.t_asymp75_Trlr [-]"; p833 "Pressure Release Time from 100% to 10% of asymptodic pressure value in [s] [TA1, TA2, TA3] export=true name=t_release10_Trlr prio=1 dataSetName=circTrlr_dummy dataClassType=circTrlr dataClassName=circTrlr unit='-' description='Pressure Release Time from 100% to 10% of asymptodic pressure value in [s] [TA1, TA2, TA3]': brkCircuitTrlr.t_release10_Trlr [-]"; p834 "Dimension Power Map [dp , om] export=true name=dim_PmechMap prio=1 dataSetName=com_dummy dataClassType=com dataClassName=com  unit='-' description='Dimension PowerMap [dp , om] ': compressor.dim_PmechMap [-]"; p835 "Dimension Volume Flow Map [dp , om] export=true name=dim_QnMap prio=1 dataSetName=com_dummy dataClassType=com dataClassName=com  unit='-' description='Dimension Volume Flow Map [dp , om] ': compressor.dim_QnMap [-]"; p836 "Dimension Temperature [dp , om] export=true name=dim_ToutMap prio=1 dataSetName=com_dummy dataClassType=com dataClassName=com  unit='-' description='Dimension Temperature Map [dp , om] ': compressor.dim_ToutMap [-]"; p837 "Pmech-om-dp Map (kW , rpm, dp) [kW] export=true name=Pmech_Map_kW prio=1 dataSetName=com_dummy dataClassType=com dataClassName=com  unit='kW' description='Pmech-om-dp Map (kW , rpm, dp) [kW]': compressor.Pmech_Map_kW [-]"; p838 "Mechanical Power Map x-Axis Compressor Speed [rpm] export=true name=Pmech_x_om_rpm prio=1 dataSetName=com_dummy dataClassType=com dataClassName=com  unit='rpm' description='Mechanical Power Map x-Axis Compressor Speed [rpm] ': compressor.Pmech_x_om_rpm [-]"; p839 "Mechanical Power Map y-Axis Compressor Pressure Drop [bar] export=true name=Pmech_y_dp_bar prio=1 dataSetName=com_dummy dataClassType=com dataClassName=com  unit='bar' description='Mechanical Power   Map y-Axis Compressor Pressure Drop [bar]': compressor.Pmech_y_dp_bar [-]"; p840 "Qn-om-dp Map (degC , rpm, dp) [degC] export=true name=Qn_Map_l_min prio=1 dataSetName=com_dummy dataClassType=com dataClassName=com  unit='l/min' description='Qn-om-dp Map (degC , rpm, dp) [degC] ': compressor.Qn_Map_l_min [-]"; p841 "Volume Flow Map x-Axis Compressor Speed [rpm] export=true name=Qn_x_om_rpm prio=1 dataSetName=com_dummy dataClassType=com dataClassName=com  unit='rpm' description='Volume Flow Map x-Axis Compressor Speed [rpm] ': compressor.Qn_x_om_rpm [-]"; p842 "Volume Flow Map y-Axis Compressor Pressure Drop [bar] export=true name=Qn_y_dp_bar prio=1 dataSetName=com_dummy dataClassType=com dataClassName=com  unit='bar' description='Volume Flow Map y-Axis Compressor Pressure Drop [bar]': compressor.Qn_y_dp_bar [-]"; p843 "Tout-om-dp Map (degC , rpm, dp) [degC] export=true name=Tout_Map_degC prio=1 dataSetName=com_dummy dataClassType=com dataClassName=com  unit='deg C' description='Tout-om-dp Map (degC , rpm, dp) [degC]': compressor.Tout_Map_degC [-]"; p844 "Temperature Map x-Axis Compressor Speed [rpm] export=true name=Tout_x_om_rpm prio=1 dataSetName=com_dummy dataClassType=com dataClassName=com  unit='rpm' description='Temperature Map x-Axis Compressor Speed [rpm] ': compressor.Tout_x_om_rpm [-]"; p845 "Temperature Map y-Axis Compressor Pressure Drop [bar] export=true name=Tout_y_dp_bar prio=1 dataSetName=com_dummy dataClassType=com dataClassName=com  unit='bar' description='Temperature  Map y-Axis Compressor Pressure Drop [bar]': compressor.Tout_y_dp_bar [-]"; p846 "Axle Loads Tractor export=true name=axleLoadTractor_kg prio=1 dataSetName=veh_dummy dataClassType=veh dataClassName=veh unit=kg description='Axle Loads Tractor': pne3d_veh_Param.axleLoadTractor_kg [-]"; p847 "Axle Loads Trailer export=true name=axleLoadTrailer_kg prio=1 dataSetName=veh_dummy dataClassType=veh dataClassName=veh unit=kg description='Axle Loads Trailer': pne3d_veh_Param.axleLoadTrailer_kg [-]"; p848 "Axle spring types of tractor 0->undefined, 1->air, 2->steel export=true name=AxleSpringType prio=1 dataSetName=veh_dummy dataClassType=veh dataClassName=veh unit='' description='Axle spring types of tractor 0->undefined, 1->air, 2->steel': pne3d_veh_Param.AxleSpringType [-]"; p849 "pAppCyl Tractor Axles [A1, A2, A3, A4] [bar] export=true name=pAppCyl_Tractor prio=1 dataSetName=veh_dummy dataClassType=veh dataClassName=veh unit='bar' description='pAppCyl Tractor Axles [A1, A2, A3, A4] [bar]': pne3d_veh_Param.pAppCyl_Tractor [-]"; p850 "pAppCyl Trailer Axles [TA1, TA2, TA3] [bar] export=true name=pAppCyl_Trailer prio=1 dataSetName=veh_dummy dataClassType=veh dataClassName=veh unit='bar' description='pAppCyl Trailer Axles [TA1, TA2, TA3] [bar]': pne3d_veh_Param.pAppCyl_Trailer [-]"; p851 "rdyn's of Vehicle/Tractor [A1,A2,A3,A4] export=true name=rdynTractor prio=1 dataSetName=veh_dummy dataClassType=veh dataClassName=veh unit=mm description='Tractor rDyn': pne3d_veh_Param.rdynTractor [-]"; p852 "rdyn's of Trailer [A1,A2,A3] export=true name=rdynTrailer prio=1 dataSetName=veh_dummy dataClassType=veh dataClassName=veh unit=mm description='Trailer rDyn': pne3d_veh_Param.rdynTrailer [-]"; p853 "Axle Loads Trailer export=true name=axleLoadTrailer02_kg prio=1 dataSetName=veh_dummy dataClassType=veh dataClassName=veh unit=kg description='Axle Loads Trailer02': pne3d_veh_Param_Roadtrain.axleLoadTrailer02_kg [-]"; p854 "application pressure of trailer axles [A1, A2, A3, A4, A5, A6] [bar] export=true name=pAppCyl_Trailer02 prio=1 dataSetName=veh_dummy dataClassType=veh dataClassName=veh unit='bar' description='application pressure of trailer axles [A1, A2, A3, A4, A5, A6]  [bar]': pne3d_veh_Param_Roadtrain.pAppCyl_Trailer02 [-]"; p855 "rdyn's of Trailer02 [A1,A2,A3, A4, A5, A6] export=true name=rdynTrailer02 prio=1 dataSetName=veh_dummy dataClassType=veh dataClassName=veh unit=mm description='Trailer02 rDyn': pne3d_veh_Param_Roadtrain.rdynTrailer02 [-]"; p856 "initial wear for each axle [A1,A2,A3,A4,Tr1,Tr2,Tr3] export=true name=initial_wear prio=1 dataSetName=default dataClassType=initialTemperatures dataClassName=initialTemperatures unit='%' description='initial wear of brakes': T_initial_brakes_Param.initial_wear [-]"; p857 "initial brake temperatures for each axle [A1,A2,A3,A4,Tr1,Tr2,Tr3] export=true name=T_initial_brakes prio=1 dataSetName=default dataClassType=initialTemperatures dataClassName=initialTemperatures unit=C description='initial temperatures of brakes': T_initial_brakes_Param.T_initial_brakes [-]"
      mask help: Generated by SimulationX 4.0.5.60286 x64
      mask init:
      | if ~isempty(initCmd), try, evalin('base', initCmd); end, end
      mask Display: disp('pne_pne3d_generic_std_sf'); port_label('input', 1, 'ebs_AdditionalAxle_left_pDmd'); port_label('input', 2, 'ebs_AdditionalAxle_left_setABS'); port_label('input', 3, 'ebs_AdditionalAxle_right_pDmd'); port_label('input', 4, 'ebs_AdditionalAxle_right_setABS'); port_label('input', 5, 'ebs_ESCsens_y_acceleration'); port_label('input', 6, 'ebs_FrontAxle_left_pDmd'); port_label('input', 7, 'ebs_FrontAxle_left_setABS'); port_label('input', 8, 'ebs_FrontAxle_right_pDmd'); port_label('input', 9, 'ebs_FrontAxle_right_setABS'); port_label('input', 10, 'ebs_RearAxle_left_pDmd'); port_label('input', 11, 'ebs_RearAxle_left_setABS'); port_label('input', 12, 'ebs_RearAxle_right_pDmd'); port_label('input', 13, 'ebs_RearAxle_right_setABS'); port_label('input', 14, 'ebs_sBSP_stABSInValve_Addl_Left'); port_label('input', 15, 'ebs_sBSP_stABSInValve_Addl_Right'); port_label('input', 16, 'ebs_sBSP_stABSInValve_Front_Left'); port_label('input', 17, 'ebs_sBSP_stABSInValve_Front_Right'); port_label('input', 18, 'ebs_sBSP_stABSInValve_RCMax_Front'); port_label('input', 19, 'ebs_sBSP_stABSInValve_RCMax_Rear'); port_label('input', 20, 'ebs_sBSP_stABSInValve_Rear_Left'); port_label('input', 21, 'ebs_sBSP_stABSInValve_Rear_Right'); port_label('input', 22, 'ebs_sBSP_stABSOutValve_Addl_Left'); port_label('input', 23, 'ebs_sBSP_stABSOutValve_Addl_Right'); port_label('input', 24, 'ebs_sBSP_stABSOutValve_Front_Left'); port_label('input', 25, 'ebs_sBSP_stABSOutValve_Front_Right'); port_label('input', 26, 'ebs_sBSP_stABSOutValve_RCMax_Front'); port_label('input', 27, 'ebs_sBSP_stABSOutValve_RCMax_Rear'); port_label('input', 28, 'ebs_sBSP_stABSOutValve_Rear_Left'); port_label('input', 29, 'ebs_sBSP_stABSOutValve_Rear_Right'); port_label('input', 30, 'ebs_sBSP_stAPCVBuValve'); port_label('input', 31, 'ebs_sBSP_stAPCVInValve'); port_label('input', 32, 'ebs_sBSP_stAPCVOutValve'); port_label('input', 33, 'ebs_sBSP_stAtcCutOffValve'); port_label('input', 34, 'ebs_sBSP_stAxmoBuValve'); port_label('input', 35, 'ebs_sBSP_stAxmoInValve_Rear_Left'); port_label('input', 36, 'ebs_sBSP_stAxmoInValve_Rear_Right'); port_label('input', 37, 'ebs_sBSP_stAxmoOutValve_Rear_Left'); port_label('input', 38, 'ebs_sBSP_stAxmoOutValve_Rear_Right'); port_label('input', 39, 'ebs_sBSP_stCMaxBuValve'); port_label('input', 40, 'ebs_sBSP_stCMaxInValve_Rear_Left'); port_label('input', 41, 'ebs_sBSP_stCMaxInValve_Rear_Right'); port_label('input', 42, 'ebs_sBSP_stCMaxOutValve_Rear_Left'); port_label('input', 43, 'ebs_sBSP_stCMaxOutValve_Rear_Right'); port_label('input', 44, 'ebs_sBSP_stRCMaxInValve_Front'); port_label('input', 45, 'ebs_sBSP_stRCMaxInValve_Rear'); port_label('input', 46, 'ebs_sBSP_stRCMaxOutValve_Front'); port_label('input', 47, 'ebs_sBSP_stRCMaxOutValve_Rear'); port_label('input', 48, 'ebs_sBSP_stTCVBuValve'); port_label('input', 49, 'ebs_sBSP_stTCVInValve'); port_label('input', 50, 'ebs_sBSP_stTCVOutValve'); port_label('input', 51, 'ebs_sil_AAle_force'); port_label('input', 52, 'ebs_sil_AAle_vel'); port_label('input', 53, 'ebs_sil_AAri_force'); port_label('input', 54, 'ebs_sil_AAri_vel'); port_label('input', 55, 'ebs_sil_FAle_force'); port_label('input', 56, 'ebs_sil_FAle_vel'); port_label('input', 57, 'ebs_sil_FAri_force'); port_label('input', 58, 'ebs_sil_FAri_vel'); port_label('input', 59, 'ebs_sil_RAle_force'); port_label('input', 60, 'ebs_sil_RAle_vel'); port_label('input', 61, 'ebs_sil_RAri_force'); port_label('input', 62, 'ebs_sil_RAri_vel'); port_label('input', 63, 'ebs_st3by2_First'); port_label('input', 64, 'ebs_st3by2_Second'); port_label('input', 65, 'ebs_TCV_pDmd'); port_label('input', 66, 'Failure_electric_circuit_AA'); port_label('input', 67, 'Failure_electric_circuit_FA'); port_label('input', 68, 'Failure_electric_circuit_RA'); port_label('input', 69, 'Failure_pneumatic_circuit_FA'); port_label('input', 70, 'Failure_pneumatic_circuit_RA'); port_label('input', 71, 'pneAux_A1_Le_Rq'); port_label('input', 72, 'pneAux_A1_LoLi_Rq'); port_label('input', 73, 'pneAux_A1_Ri_Rq'); port_label('input', 74, 'pneAux_A2_Le_Rq'); port_label('input', 75, 'pneAux_A2_LoLi_Rq'); port_label('input', 76, 'pneAux_A2_Ri_Rq'); port_label('input', 77, 'pneAux_A3_Le_Rq'); port_label('input', 78, 'pneAux_A3_LoLi_Rq'); port_label('input', 79, 'pneAux_A3_Ri_Rq'); port_label('input', 80, 'pneAux_Axle1_load'); port_label('input', 81, 'pneAux_Axle2_load'); port_label('input', 82, 'pneAux_Axle3_load'); port_label('input', 83, 'pneAux_Axle4_load'); port_label('input', 84, 'pneAux_Drs_Rq'); port_label('input', 85, 'pneAux_EAPU_overrun'); port_label('input', 86, 'pneAux_pSoll_TCV_p43'); port_label('input', 87, 'pneAux_pSollPkBrk'); port_label('input', 88, 'pneAux_TCV_pDmd_Front_Left'); port_label('input', 89, 'pneAux_TCV_pDmd_Front_Right'); port_label('input', 90, 'pneAux_TCV_pDmd_Rear_Left'); port_label('input', 91, 'pneAux_TCV_pDmd_Rear_Right'); port_label('input', 92, 'pneAux_trailerAxle1_left_stABSInValve'); port_label('input', 93, 'pneAux_trailerAxle1_left_stABSOutValve'); port_label('input', 94, 'pneAux_trailerAxle1_load'); port_label('input', 95, 'pneAux_trailerAxle1_right_stABSInValve'); port_label('input', 96, 'pneAux_trailerAxle1_right_stABSOutValve'); port_label('input', 97, 'pneAux_trailerAxle2_left_stABSInValve'); port_label('input', 98, 'pneAux_trailerAxle2_left_stABSOutValve'); port_label('input', 99, 'pneAux_trailerAxle2_load'); port_label('input', 100, 'pneAux_trailerAxle2_right_stABSInValve'); port_label('input', 101, 'pneAux_trailerAxle2_right_stABSOutValve'); port_label('input', 102, 'pneAux_trailerAxle3_left_stABSInValve'); port_label('input', 103, 'pneAux_trailerAxle3_left_stABSOutValve'); port_label('input', 104, 'pneAux_trailerAxle3_load'); port_label('input', 105, 'pneAux_trailerAxle3_right_stABSInValve'); port_label('input', 106, 'pneAux_trailerAxle3_right_stABSOutValve'); port_label('input', 107, 'env_air_frontVel'); port_label('input', 108, 'env_pressure'); port_label('input', 109, 'env_Temperature'); port_label('input', 110, 'pne_brk_AirCompressor_angAcc'); port_label('input', 111, 'pne_brk_AirCompressor_angPos'); port_label('input', 112, 'pne_brk_AirCompressor_angVel'); port_label('input', 113, 'pne_brk_AirConsumpEng_mdot'); port_label('input', 114, 'pne_brk_AirConsumpRet_mdot'); port_label('input', 115, 'pne_brk_AirConsumpTx_mdot'); port_label('input', 116, 'pne_brk_Axle1_left_angAcc'); port_label('input', 117, 'pne_brk_Axle1_left_angPos'); port_label('input', 118, 'pne_brk_Axle1_left_angVel'); port_label('input', 119, 'pne_brk_Axle1_right_angAcc'); port_label('input', 120, 'pne_brk_Axle1_right_angPos'); port_label('input', 121, 'pne_brk_Axle1_right_angVel'); port_label('input', 122, 'pne_brk_Axle2_left_angAcc'); port_label('input', 123, 'pne_brk_Axle2_left_angPos'); port_label('input', 124, 'pne_brk_Axle2_left_angVel'); port_label('input', 125, 'pne_brk_Axle2_right_angAcc'); port_label('input', 126, 'pne_brk_Axle2_right_angPos'); port_label('input', 127, 'pne_brk_Axle2_right_angVel'); port_label('input', 128, 'pne_brk_Axle3_left_angAcc'); port_label('input', 129, 'pne_brk_Axle3_left_angPos'); port_label('input', 130, 'pne_brk_Axle3_left_angVel'); port_label('input', 131, 'pne_brk_Axle3_right_angAcc'); port_label('input', 132, 'pne_brk_Axle3_right_angPos'); port_label('input', 133, 'pne_brk_Axle3_right_angVel'); port_label('input', 134, 'pne_brk_Axle4_left_angAcc'); port_label('input', 135, 'pne_brk_Axle4_left_angPos'); port_label('input', 136, 'pne_brk_Axle4_left_angVel'); port_label('input', 137, 'pne_brk_Axle4_right_angAcc'); port_label('input', 138, 'pne_brk_Axle4_right_angPos'); port_label('input', 139, 'pne_brk_Axle4_right_angVel'); port_label('input', 140, 'pne_brk_CompressorInlet_massfracH2O'); port_label('input', 141, 'pne_brk_CompressorInlet_pressure'); port_label('input', 142, 'pne_brk_CompressorInlet_Temperature'); port_label('input', 143, 'pne_brk_PowerBoost_mdot'); port_label('input', 144, 'pne_brk_TrailerAxle1_left_angAcc'); port_label('input', 145, 'pne_brk_TrailerAxle1_left_angPos'); port_label('input', 146, 'pne_brk_TrailerAxle1_left_angVel'); port_label('input', 147, 'pne_brk_TrailerAxle1_right_angAcc'); port_label('input', 148, 'pne_brk_TrailerAxle1_right_angPos'); port_label('input', 149, 'pne_brk_TrailerAxle1_right_angVel'); port_label('input', 150, 'pne_brk_TrailerAxle2_left_angAcc'); port_label('input', 151, 'pne_brk_TrailerAxle2_left_angPos'); port_label('input', 152, 'pne_brk_TrailerAxle2_left_angVel'); port_label('input', 153, 'pne_brk_TrailerAxle2_right_angAcc'); port_label('input', 154, 'pne_brk_TrailerAxle2_right_angPos'); port_label('input', 155, 'pne_brk_TrailerAxle2_right_angVel'); port_label('input', 156, 'pne_brk_TrailerAxle3_left_angAcc'); port_label('input', 157, 'pne_brk_TrailerAxle3_left_angPos'); port_label('input', 158, 'pne_brk_TrailerAxle3_left_angVel'); port_label('input', 159, 'pne_brk_TrailerAxle3_right_angAcc'); port_label('input', 160, 'pne_brk_TrailerAxle3_right_angPos'); port_label('input', 161, 'pne_brk_TrailerAxle3_right_angVel'); port_label('output', 1, 'pne_AirConsumptionFlow_AirSuspension'); port_label('output', 2, 'pne_AirConsumptionFlow_auxiliaries'); port_label('output', 3, 'pne_AirConsumptionFlow_doors'); port_label('output', 4, 'pne_AirConsumptionFlow_EnduranceBrakes'); port_label('output', 5, 'pne_AirConsumptionFlow_engine'); port_label('output', 6, 'pne_AirConsumptionFlow_gearbox'); port_label('output', 7, 'pne_AirConsumptionFlow_leakage'); port_label('output', 8, 'pne_AirConsumptionFlow_PowerBoost'); port_label('output', 9, 'pne_AirConsumptionFlow_SCR'); port_label('output', 10, 'pne_brk_AirCompressor_delivery'); port_label('output', 11, 'pne_brk_Axle1_BrakingPower'); port_label('output', 12, 'pne_brk_Axle1_left_kvT'); port_label('output', 13, 'pne_brk_Axle1_left_sPad_sum'); port_label('output', 14, 'pne_brk_Axle1_left_Tcooldown'); port_label('output', 15, 'pne_brk_Axle1_left_Tfriction'); port_label('output', 16, 'pne_brk_Axle1_left_torque_grinding'); port_label('output', 17, 'pne_brk_Axle1_right_kvT'); port_label('output', 18, 'pne_brk_Axle1_right_sPad_sum'); port_label('output', 19, 'pne_brk_Axle1_right_Tcooldown'); port_label('output', 20, 'pne_brk_Axle1_right_Tfriction'); port_label('output', 21, 'pne_brk_Axle1_right_torque_grinding'); port_label('output', 22, 'pne_brk_Axle1Brake_Fcyl'); port_label('output', 23, 'pne_brk_Axle1Brake_left_pRel'); port_label('output', 24, 'pne_brk_Axle1Brake_right_pRel'); port_label('output', 25, 'pne_brk_Axle1Brake_stroke'); port_label('output', 26, 'pne_brk_Axle1Brake_Vol'); port_label('output', 27, 'pne_brk_Axle2_BrakingPower'); port_label('output', 28, 'pne_brk_Axle2_left_kvT'); port_label('output', 29, 'pne_brk_Axle2_left_sPad_sum'); port_label('output', 30, 'pne_brk_Axle2_left_Tcooldown'); port_label('output', 31, 'pne_brk_Axle2_left_Tfriction'); port_label('output', 32, 'pne_brk_Axle2_left_torque_grinding'); port_label('output', 33, 'pne_brk_Axle2_right_kvT'); port_label('output', 34, 'pne_brk_Axle2_right_sPad_sum'); port_label('output', 35, 'pne_brk_Axle2_right_Tcooldown'); port_label('output', 36, 'pne_brk_Axle2_right_Tfriction'); port_label('output', 37, 'pne_brk_Axle2_right_torque_grinding'); port_label('output', 38, 'pne_brk_Axle2Brake_Fcyl'); port_label('output', 39, 'pne_brk_Axle2Brake_left_pRel'); port_label('output', 40, 'pne_brk_Axle2Brake_right_pRel'); port_label('output', 41, 'pne_brk_Axle2Brake_stroke'); port_label('output', 42, 'pne_brk_Axle2Brake_Vol'); port_label('output', 43, 'pne_brk_Axle3_BrakingPower'); port_label('output', 44, 'pne_brk_Axle3_left_kvT'); port_label('output', 45, 'pne_brk_Axle3_left_sPad_sum'); port_label('output', 46, 'pne_brk_Axle3_left_Tcooldown'); port_label('output', 47, 'pne_brk_Axle3_left_Tfriction'); port_label('output', 48, 'pne_brk_Axle3_left_torque_grinding'); port_label('output', 49, 'pne_brk_Axle3_right_kvT'); port_label('output', 50, 'pne_brk_Axle3_right_sPad_sum'); port_label('output', 51, 'pne_brk_Axle3_right_Tcooldown'); port_label('output', 52, 'pne_brk_Axle3_right_Tfriction'); port_label('output', 53, 'pne_brk_Axle3_right_torque_grinding'); port_label('output', 54, 'pne_brk_Axle3Brake_Fcyl'); port_label('output', 55, 'pne_brk_Axle3Brake_left_pRel'); port_label('output', 56, 'pne_brk_Axle3Brake_right_pRel'); port_label('output', 57, 'pne_brk_Axle3Brake_stroke'); port_label('output', 58, 'pne_brk_Axle3Brake_Vol'); port_label('output', 59, 'pne_brk_Axle4_BrakingPower'); port_label('output', 60, 'pne_brk_Axle4_left_kvT'); port_label('output', 61, 'pne_brk_Axle4_left_sPad_sum'); port_label('output', 62, 'pne_brk_Axle4_left_Tcooldown'); port_label('output', 63, 'pne_brk_Axle4_left_Tfriction'); port_label('output', 64, 'pne_brk_Axle4_left_torque_grinding'); port_label('output', 65, 'pne_brk_Axle4_right_kvT'); port_label('output', 66, 'pne_brk_Axle4_right_sPad_sum'); port_label('output', 67, 'pne_brk_Axle4_right_Tcooldown'); port_label('output', 68, 'pne_brk_Axle4_right_Tfriction'); port_label('output', 69, 'pne_brk_Axle4_right_torque_grinding'); port_label('output', 70, 'pne_brk_Axle4Brake_Fcyl'); port_label('output', 71, 'pne_brk_Axle4Brake_left_pRel'); port_label('output', 72, 'pne_brk_Axle4Brake_right_pRel'); port_label('output', 73, 'pne_brk_Axle4Brake_stroke'); port_label('output', 74, 'pne_brk_Axle4Brake_Vol'); port_label('output', 75, 'pne_brk_CompOut_Temp'); port_label('output', 76, 'pne_brk_CoolingPipe_pRel'); port_label('output', 77, 'pne_brk_CoolingPipe_Temp'); port_label('output', 78, 'pne_brk_EAPU_pRel'); port_label('output', 79, 'pne_brk_EAPU_Temp'); port_label('output', 80, 'pne_brk_TrailerAxle1_BrakingPower'); port_label('output', 81, 'pne_brk_TrailerAxle1_left_kvT'); port_label('output', 82, 'pne_brk_TrailerAxle1_left_sPad_sum'); port_label('output', 83, 'pne_brk_TrailerAxle1_left_Tcooldown'); port_label('output', 84, 'pne_brk_TrailerAxle1_left_Tfriction'); port_label('output', 85, 'pne_brk_TrailerAxle1_left_Tinterior'); port_label('output', 86, 'pne_brk_TrailerAxle1_left_torque_grinding'); port_label('output', 87, 'pne_brk_TrailerAxle1_right_kvT'); port_label('output', 88, 'pne_brk_TrailerAxle1_right_sPad_sum'); port_label('output', 89, 'pne_brk_TrailerAxle1_right_Tcooldown'); port_label('output', 90, 'pne_brk_TrailerAxle1_right_Tfriction'); port_label('output', 91, 'pne_brk_TrailerAxle1_right_Tinterior'); port_label('output', 92, 'pne_brk_TrailerAxle1_right_torque_grinding'); port_label('output', 93, 'pne_brk_TrailerAxle1Brake_Fcyl'); port_label('output', 94, 'pne_brk_TrailerAxle1Brake_left_pRel'); port_label('output', 95, 'pne_brk_TrailerAxle1Brake_right_pRel'); port_label('output', 96, 'pne_brk_TrailerAxle1Brake_stroke'); port_label('output', 97, 'pne_brk_TrailerAxle1Brake_Vol'); port_label('output', 98, 'pne_brk_TrailerAxle2_BrakingPower'); port_label('output', 99, 'pne_brk_TrailerAxle2_left_kvT'); port_label('output', 100, 'pne_brk_TrailerAxle2_left_sPad_sum'); port_label('output', 101, 'pne_brk_TrailerAxle2_left_Tcooldown'); port_label('output', 102, 'pne_brk_TrailerAxle2_left_Tfriction'); port_label('output', 103, 'pne_brk_TrailerAxle2_left_Tinterior'); port_label('output', 104, 'pne_brk_TrailerAxle2_left_torque_grinding'); port_label('output', 105, 'pne_brk_TrailerAxle2_right_kvT'); port_label('output', 106, 'pne_brk_TrailerAxle2_right_sPad_sum'); port_label('output', 107, 'pne_brk_TrailerAxle2_right_Tcooldown'); port_label('output', 108, 'pne_brk_TrailerAxle2_right_Tfriction'); port_label('output', 109, 'pne_brk_TrailerAxle2_right_Tinterior'); port_label('output', 110, 'pne_brk_TrailerAxle2_right_torque_grinding'); port_label('output', 111, 'pne_brk_TrailerAxle2Brake_Fcyl'); port_label('output', 112, 'pne_brk_TrailerAxle2Brake_left_pRel'); port_label('output', 113, 'pne_brk_TrailerAxle2Brake_right_pRel'); port_label('output', 114, 'pne_brk_TrailerAxle2Brake_stroke'); port_label('output', 115, 'pne_brk_TrailerAxle2Brake_Vol'); port_label('output', 116, 'pne_brk_TrailerAxle3_BrakingPower'); port_label('output', 117, 'pne_brk_TrailerAxle3_left_kvT'); port_label('output', 118, 'pne_brk_TrailerAxle3_left_sPad_sum'); port_label('output', 119, 'pne_brk_TrailerAxle3_left_Tcooldown'); port_label('output', 120, 'pne_brk_TrailerAxle3_left_Tfriction'); port_label('output', 121, 'pne_brk_TrailerAxle3_left_Tinterior'); port_label('output', 122, 'pne_brk_TrailerAxle3_left_torque_grinding'); port_label('output', 123, 'pne_brk_TrailerAxle3_right_kvT'); port_label('output', 124, 'pne_brk_TrailerAxle3_right_sPad_sum'); port_label('output', 125, 'pne_brk_TrailerAxle3_right_Tcooldown'); port_label('output', 126, 'pne_brk_TrailerAxle3_right_Tfriction'); port_label('output', 127, 'pne_brk_TrailerAxle3_right_Tinterior'); port_label('output', 128, 'pne_brk_TrailerAxle3_right_torque_grinding'); port_label('output', 129, 'pne_brk_TrailerAxle3Brake_Fcyl'); port_label('output', 130, 'pne_brk_TrailerAxle3Brake_left_pRel'); port_label('output', 131, 'pne_brk_TrailerAxle3Brake_right_pRel'); port_label('output', 132, 'pne_brk_TrailerAxle3Brake_stroke'); port_label('output', 133, 'pne_brk_TrailerAxle3Brake_Vol'); port_label('output', 134, 'pne_brk_V1_Temp'); port_label('output', 135, 'pne_brk_V2_Temp'); port_label('output', 136, 'pne_brk_V3_pRel'); port_label('output', 137, 'pne_brk_V3_Temp'); port_label('output', 138, 'pne_brk_V4_Temp'); port_label('output', 139, 'pne_brk_V5_pRel'); port_label('output', 140, 'pne_brk_V5_Temp'); port_label('output', 141, 'pne_brk_V6_pRel'); port_label('output', 142, 'pne_brk_V6_Temp'); port_label('output', 143, 'pne_brk_V7_Temp'); port_label('output', 144, 'pne_brk_V8_pRel'); port_label('output', 145, 'pne_brk_V8_Temp'); port_label('output', 146, 'pne_brk_Vsup_pRel'); port_label('output', 147, 'pne_brk_Vsup_Temp'); port_label('output', 148, 'pne_brk_VTrailer_Temp'); port_label('output', 149, 'pne_brk_AirCompressor_torque'); port_label('output', 150, 'pne_brk_AirConsumpEng_massfracH2O'); port_label('output', 151, 'pne_brk_AirConsumpEng_pressure'); port_label('output', 152, 'pne_brk_AirConsumpEng_Temperature'); port_label('output', 153, 'pne_brk_AirConsumpRet_massfracH2O'); port_label('output', 154, 'pne_brk_AirConsumpRet_pressure'); port_label('output', 155, 'pne_brk_AirConsumpRet_Temperature'); port_label('output', 156, 'pne_brk_AirConsumpTx_massfracH2O'); port_label('output', 157, 'pne_brk_AirConsumpTx_pressure'); port_label('output', 158, 'pne_brk_AirConsumpTx_Temperature'); port_label('output', 159, 'pne_brk_Axle1_left_torque'); port_label('output', 160, 'pne_brk_Axle1_right_torque'); port_label('output', 161, 'pne_brk_Axle2_left_torque'); port_label('output', 162, 'pne_brk_Axle2_right_torque'); port_label('output', 163, 'pne_brk_Axle3_left_torque'); port_label('output', 164, 'pne_brk_Axle3_right_torque'); port_label('output', 165, 'pne_brk_Axle4_left_torque'); port_label('output', 166, 'pne_brk_Axle4_right_torque'); port_label('output', 167, 'pne_brk_CompressorInlet_mdot'); port_label('output', 168, 'pne_brk_PowerBoost_massfracH2O'); port_label('output', 169, 'pne_brk_PowerBoost_pressure'); port_label('output', 170, 'pne_brk_PowerBoost_Temperature'); port_label('output', 171, 'pne_brk_TrailerAxle1_left_torque'); port_label('output', 172, 'pne_brk_TrailerAxle1_right_torque'); port_label('output', 173, 'pne_brk_TrailerAxle2_left_torque'); port_label('output', 174, 'pne_brk_TrailerAxle2_right_torque'); port_label('output', 175, 'pne_brk_TrailerAxle3_left_torque'); port_label('output', 176, 'pne_brk_TrailerAxle3_right_torque'); port_label('output', 177, 'pne_brk_Actual_Pressure_AL'); port_label('output', 178, 'pne_brk_Actual_Pressure_AR'); port_label('output', 179, 'pne_brk_Actual_Pressure_FA'); port_label('output', 180, 'pne_brk_Actual_Pressure_FOPB'); port_label('output', 181, 'pne_brk_Actual_Pressure_Front'); port_label('output', 182, 'pne_brk_Actual_Pressure_Rear'); port_label('output', 183, 'pne_brk_Actual_Pressure_RL'); port_label('output', 184, 'pne_brk_Actual_Pressure_RR'); port_label('output', 185, 'pne_brk_Actual_Pressure_TCV'); port_label('output', 186, 'pne_brk_AdditionalAxle_AxMo_left_rotVel'); port_label('output', 187, 'pne_brk_AdditionalAxle_AxMo_right_rotVel'); port_label('output', 188, 'pne_brk_AdditionalAxle_left_pAct'); port_label('output', 189, 'pne_brk_AdditionalAxle_left_rotVel'); port_label('output', 190, 'pne_brk_AdditionalAxle_right_pAct'); port_label('output', 191, 'pne_brk_AdditionalAxle_right_rotVel'); port_label('output', 192, 'pne_brk_Axle1_BrakingForce_at8p5bar'); port_label('output', 193, 'pne_brk_Axle1_left_Tinterior'); port_label('output', 194, 'pne_brk_Axle1_right_Tinterior'); port_label('output', 195, 'pne_brk_Axle1_torque_sns'); port_label('output', 196, 'pne_brk_Axle2_BrakingForce_at8p5bar'); port_label('output', 197, 'pne_brk_Axle2_left_Tinterior'); port_label('output', 198, 'pne_brk_Axle2_right_Tinterior'); port_label('output', 199, 'pne_brk_Axle2_torque_sns'); port_label('output', 200, 'pne_brk_Axle3_BrakingForce_at8p5bar'); port_label('output', 201, 'pne_brk_Axle3_left_Tinterior'); port_label('output', 202, 'pne_brk_Axle3_right_Tinterior'); port_label('output', 203, 'pne_brk_Axle3_torque_sns'); port_label('output', 204, 'pne_brk_Axle4_BrakingForce_at8p5bar'); port_label('output', 205, 'pne_brk_Axle4_left_Tinterior'); port_label('output', 206, 'pne_brk_Axle4_right_Tinterior'); port_label('output', 207, 'pne_brk_Axle4_torque_sns'); port_label('output', 208, 'pne_brk_BrkWearAALt'); port_label('output', 209, 'pne_brk_BrkWearAARt'); port_label('output', 210, 'pne_brk_BrkWearFA1Lt'); port_label('output', 211, 'pne_brk_BrkWearFA1Rt'); port_label('output', 212, 'pne_brk_BrkWearFA2Lt'); port_label('output', 213, 'pne_brk_BrkWearFA2Rt'); port_label('output', 214, 'pne_brk_BrkWearRA1Lt'); port_label('output', 215, 'pne_brk_BrkWearRA1Rt'); port_label('output', 216, 'pne_brk_BrkWearRA2Lt'); port_label('output', 217, 'pne_brk_BrkWearRA2Rt'); port_label('output', 218, 'pne_brk_CompON'); port_label('output', 219, 'pne_brk_FrontAxle_left_rotVel'); port_label('output', 220, 'pne_brk_FrontAxle_pAct'); port_label('output', 221, 'pne_brk_FrontAxle_right_rotVel'); port_label('output', 222, 'pne_brk_pRelPkBrk'); port_label('output', 223, 'pne_brk_RearAxle_left_pAct'); port_label('output', 224, 'pne_brk_RearAxle_left_rotVel'); port_label('output', 225, 'pne_brk_RearAxle_right_pAct'); port_label('output', 226, 'pne_brk_RearAxle_right_rotVel'); port_label('output', 227, 'pne_brk_reg_active'); port_label('output', 228, 'pne_brk_rotVel_al'); port_label('output', 229, 'pne_brk_rotVel_ar'); port_label('output', 230, 'pne_brk_rotVel_fl'); port_label('output', 231, 'pne_brk_rotVel_fr'); port_label('output', 232, 'pne_brk_rotVel_rl'); port_label('output', 233, 'pne_brk_rotVel_rr'); port_label('output', 234, 'pne_brk_rotVel_t1l'); port_label('output', 235, 'pne_brk_rotVel_t1r'); port_label('output', 236, 'pne_brk_rotVel_t2l'); port_label('output', 237, 'pne_brk_rotVel_t2r'); port_label('output', 238, 'pne_brk_rotVel_t3l'); port_label('output', 239, 'pne_brk_rotVel_t3r'); port_label('output', 240, 'pne_brk_TCV_pAct'); port_label('output', 241, 'pne_brk_Trailer_RV_Front_pAct'); port_label('output', 242, 'pne_brk_Trailer_RV_Rear_pAct'); port_label('output', 243, 'pne_brk_TrailerAxle1_BrakingForce_at8p5bar'); port_label('output', 244, 'pne_brk_TrailerAxle1_torque_sns'); port_label('output', 245, 'pne_brk_TrailerAxle2_BrakingForce_at8p5bar'); port_label('output', 246, 'pne_brk_TrailerAxle2_torque_sns'); port_label('output', 247, 'pne_brk_TrailerAxle3_BrakingForce_at8p5bar'); port_label('output', 248, 'pne_brk_TrailerAxle3_torque_sns'); port_label('output', 249, 'pne_brk_V1_pRel'); port_label('output', 250, 'pne_brk_V2_pRel'); port_label('output', 251, 'pne_brk_V4_pRel'); port_label('output', 252, 'pne_brk_V7_pRel'); port_label('output', 253, 'pne_brk_VTrailer_pRel'); port_label('output', 254, 'pne_brk_WetLvl_Cntr'); port_label('output', 255, 'pne_susp_A1_Le_Posn'); port_label('output', 256, 'pne_susp_A1_Ri_Posn'); port_label('output', 257, 'pne_susp_A2_Le_Posn'); port_label('output', 258, 'pne_susp_A2_Ri_Posn'); port_label('output', 259, 'pne_susp_A3_Le_Posn'); port_label('output', 260, 'pne_susp_A3_Ri_Posn');
  pne_AirConsumptionFlow_AirSuspension : Outport
  pne_AirConsumptionFlow_auxiliaries : Outport  Port=2
  pne_AirConsumptionFlow_doors : Outport  Port=3
  pne_AirConsumptionFlow_EnduranceBrakes : Outport  Port=4
  pne_AirConsumptionFlow_engine : Outport  Port=5
  pne_AirConsumptionFlow_gearbox : Outport  Port=6
  pne_AirConsumptionFlow_leakage : Outport  Port=7
  pne_AirConsumptionFlow_PowerBoost : Outport  Port=8
  pne_AirConsumptionFlow_SCR : Outport  Port=9
  pne_brk_AirCompressor_delivery : Outport  Port=10
  pne_brk_Axle1_BrakingPower : Outport  Port=11
  pne_brk_Axle1_left_kvT : Outport  Port=12
  pne_brk_Axle1_left_sPad_sum : Outport  Port=13
  pne_brk_Axle1_left_Tcooldown : Outport  Port=14
  pne_brk_Axle1_left_Tfriction : Outport  Port=15
  pne_brk_Axle1_left_torque_grinding : Outport  Port=16
  pne_brk_Axle1_right_kvT : Outport  Port=17
  pne_brk_Axle1_right_sPad_sum : Outport  Port=18
  pne_brk_Axle1_right_Tcooldown : Outport  Port=19
  pne_brk_Axle1_right_Tfriction : Outport  Port=20
  pne_brk_Axle1_right_torque_grinding : Outport  Port=21
  pne_brk_Axle1Brake_Fcyl : Outport  Port=22
  pne_brk_Axle1Brake_left_pRel : Outport  Port=23
  pne_brk_Axle1Brake_right_pRel : Outport  Port=24
  pne_brk_Axle1Brake_stroke : Outport  Port=25
  pne_brk_Axle1Brake_Vol : Outport  Port=26
  pne_brk_Axle2_BrakingPower : Outport  Port=27
  pne_brk_Axle2_left_kvT : Outport  Port=28
  pne_brk_Axle2_left_sPad_sum : Outport  Port=29
  pne_brk_Axle2_left_Tcooldown : Outport  Port=30
  pne_brk_Axle2_left_Tfriction : Outport  Port=31
  pne_brk_Axle2_left_torque_grinding : Outport  Port=32
  pne_brk_Axle2_right_kvT : Outport  Port=33
  pne_brk_Axle2_right_sPad_sum : Outport  Port=34
  pne_brk_Axle2_right_Tcooldown : Outport  Port=35
  pne_brk_Axle2_right_Tfriction : Outport  Port=36
  pne_brk_Axle2_right_torque_grinding : Outport  Port=37
  pne_brk_Axle2Brake_Fcyl : Outport  Port=38
  pne_brk_Axle2Brake_left_pRel : Outport  Port=39
  pne_brk_Axle2Brake_right_pRel : Outport  Port=40
  pne_brk_Axle2Brake_stroke : Outport  Port=41
  pne_brk_Axle2Brake_Vol : Outport  Port=42
  pne_brk_Axle3_BrakingPower : Outport  Port=43
  pne_brk_Axle3_left_kvT : Outport  Port=44
  pne_brk_Axle3_left_sPad_sum : Outport  Port=45
  pne_brk_Axle3_left_Tcooldown : Outport  Port=46
  pne_brk_Axle3_left_Tfriction : Outport  Port=47
  pne_brk_Axle3_left_torque_grinding : Outport  Port=48
  pne_brk_Axle3_right_kvT : Outport  Port=49
  pne_brk_Axle3_right_sPad_sum : Outport  Port=50
  pne_brk_Axle3_right_Tcooldown : Outport  Port=51
  pne_brk_Axle3_right_Tfriction : Outport  Port=52
  pne_brk_Axle3_right_torque_grinding : Outport  Port=53
  pne_brk_Axle3Brake_Fcyl : Outport  Port=54
  pne_brk_Axle3Brake_left_pRel : Outport  Port=55
  pne_brk_Axle3Brake_right_pRel : Outport  Port=56
  pne_brk_Axle3Brake_stroke : Outport  Port=57
  pne_brk_Axle3Brake_Vol : Outport  Port=58
  pne_brk_Axle4_BrakingPower : Outport  Port=59
  pne_brk_Axle4_left_kvT : Outport  Port=60
  pne_brk_Axle4_left_sPad_sum : Outport  Port=61
  pne_brk_Axle4_left_Tcooldown : Outport  Port=62
  pne_brk_Axle4_left_Tfriction : Outport  Port=63
  pne_brk_Axle4_left_torque_grinding : Outport  Port=64
  pne_brk_Axle4_right_kvT : Outport  Port=65
  pne_brk_Axle4_right_sPad_sum : Outport  Port=66
  pne_brk_Axle4_right_Tcooldown : Outport  Port=67
  pne_brk_Axle4_right_Tfriction : Outport  Port=68
  pne_brk_Axle4_right_torque_grinding : Outport  Port=69
  pne_brk_Axle4Brake_Fcyl : Outport  Port=70
  pne_brk_Axle4Brake_left_pRel : Outport  Port=71
  pne_brk_Axle4Brake_right_pRel : Outport  Port=72
  pne_brk_Axle4Brake_stroke : Outport  Port=73
  pne_brk_Axle4Brake_Vol : Outport  Port=74
  pne_brk_CompOut_Temp : Outport  Port=75
  pne_brk_CoolingPipe_pRel : Outport  Port=76
  pne_brk_CoolingPipe_Temp : Outport  Port=77
  pne_brk_EAPU_pRel : Outport  Port=78
  pne_brk_EAPU_Temp : Outport  Port=79
  pne_brk_TrailerAxle1_BrakingPower : Outport  Port=80
  pne_brk_TrailerAxle1_left_kvT : Outport  Port=81
  pne_brk_TrailerAxle1_left_sPad_sum : Outport  Port=82
  pne_brk_TrailerAxle1_left_Tcooldown : Outport  Port=83
  pne_brk_TrailerAxle1_left_Tfriction : Outport  Port=84
  pne_brk_TrailerAxle1_left_Tinterior : Outport  Port=85
  pne_brk_TrailerAxle1_left_torque_grinding : Outport  Port=86
  pne_brk_TrailerAxle1_right_kvT : Outport  Port=87
  pne_brk_TrailerAxle1_right_sPad_sum : Outport  Port=88
  pne_brk_TrailerAxle1_right_Tcooldown : Outport  Port=89
  pne_brk_TrailerAxle1_right_Tfriction : Outport  Port=90
  pne_brk_TrailerAxle1_right_Tinterior : Outport  Port=91
  pne_brk_TrailerAxle1_right_torque_grinding : Outport  Port=92
  pne_brk_TrailerAxle1Brake_Fcyl : Outport  Port=93
  pne_brk_TrailerAxle1Brake_left_pRel : Outport  Port=94
  pne_brk_TrailerAxle1Brake_right_pRel : Outport  Port=95
  pne_brk_TrailerAxle1Brake_stroke : Outport  Port=96
  pne_brk_TrailerAxle1Brake_Vol : Outport  Port=97
  pne_brk_TrailerAxle2_BrakingPower : Outport  Port=98
  pne_brk_TrailerAxle2_left_kvT : Outport  Port=99
  pne_brk_TrailerAxle2_left_sPad_sum : Outport  Port=100
  pne_brk_TrailerAxle2_left_Tcooldown : Outport  Port=101
  pne_brk_TrailerAxle2_left_Tfriction : Outport  Port=102
  pne_brk_TrailerAxle2_left_Tinterior : Outport  Port=103
  pne_brk_TrailerAxle2_left_torque_grinding : Outport  Port=104
  pne_brk_TrailerAxle2_right_kvT : Outport  Port=105
  pne_brk_TrailerAxle2_right_sPad_sum : Outport  Port=106
  pne_brk_TrailerAxle2_right_Tcooldown : Outport  Port=107
  pne_brk_TrailerAxle2_right_Tfriction : Outport  Port=108
  pne_brk_TrailerAxle2_right_Tinterior : Outport  Port=109
  pne_brk_TrailerAxle2_right_torque_grinding : Outport  Port=110
  pne_brk_TrailerAxle2Brake_Fcyl : Outport  Port=111
  pne_brk_TrailerAxle2Brake_left_pRel : Outport  Port=112
  pne_brk_TrailerAxle2Brake_right_pRel : Outport  Port=113
  pne_brk_TrailerAxle2Brake_stroke : Outport  Port=114
  pne_brk_TrailerAxle2Brake_Vol : Outport  Port=115
  pne_brk_TrailerAxle3_BrakingPower : Outport  Port=116
  pne_brk_TrailerAxle3_left_kvT : Outport  Port=117
  pne_brk_TrailerAxle3_left_sPad_sum : Outport  Port=118
  pne_brk_TrailerAxle3_left_Tcooldown : Outport  Port=119
  pne_brk_TrailerAxle3_left_Tfriction : Outport  Port=120
  pne_brk_TrailerAxle3_left_Tinterior : Outport  Port=121
  pne_brk_TrailerAxle3_left_torque_grinding : Outport  Port=122
  pne_brk_TrailerAxle3_right_kvT : Outport  Port=123
  pne_brk_TrailerAxle3_right_sPad_sum : Outport  Port=124
  pne_brk_TrailerAxle3_right_Tcooldown : Outport  Port=125
  pne_brk_TrailerAxle3_right_Tfriction : Outport  Port=126
  pne_brk_TrailerAxle3_right_Tinterior : Outport  Port=127
  pne_brk_TrailerAxle3_right_torque_grinding : Outport  Port=128
  pne_brk_TrailerAxle3Brake_Fcyl : Outport  Port=129
  pne_brk_TrailerAxle3Brake_left_pRel : Outport  Port=130
  pne_brk_TrailerAxle3Brake_right_pRel : Outport  Port=131
  pne_brk_TrailerAxle3Brake_stroke : Outport  Port=132
  pne_brk_TrailerAxle3Brake_Vol : Outport  Port=133
  pne_brk_V1_Temp : Outport  Port=134
  pne_brk_V2_Temp : Outport  Port=135
  pne_brk_V3_pRel : Outport  Port=136
  pne_brk_V3_Temp : Outport  Port=137
  pne_brk_V4_Temp : Outport  Port=138
  pne_brk_V5_pRel : Outport  Port=139
  pne_brk_V5_Temp : Outport  Port=140
  pne_brk_V6_pRel : Outport  Port=141
  pne_brk_V6_Temp : Outport  Port=142
  pne_brk_V7_Temp : Outport  Port=143
  pne_brk_V8_pRel : Outport  Port=144
  pne_brk_V8_Temp : Outport  Port=145
  pne_brk_Vsup_pRel : Outport  Port=146
  pne_brk_Vsup_Temp : Outport  Port=147
  pne_brk_VTrailer_Temp : Outport  Port=148
  pne_brk_AirCompressor_torque : Outport  Port=149
  pne_brk_AirConsumpEng_massfracH2O : Outport  Port=150
  pne_brk_AirConsumpEng_pressure : Outport  Port=151
  pne_brk_AirConsumpEng_Temperature : Outport  Port=152
  pne_brk_AirConsumpRet_massfracH2O : Outport  Port=153
  pne_brk_AirConsumpRet_pressure : Outport  Port=154
  pne_brk_AirConsumpRet_Temperature : Outport  Port=155
  pne_brk_AirConsumpTx_massfracH2O : Outport  Port=156
  pne_brk_AirConsumpTx_pressure : Outport  Port=157
  pne_brk_AirConsumpTx_Temperature : Outport  Port=158
  pne_brk_Axle1_left_torque : Outport  Port=159
  pne_brk_Axle1_right_torque : Outport  Port=160
  pne_brk_Axle2_left_torque : Outport  Port=161
  pne_brk_Axle2_right_torque : Outport  Port=162
  pne_brk_Axle3_left_torque : Outport  Port=163
  pne_brk_Axle3_right_torque : Outport  Port=164
  pne_brk_Axle4_left_torque : Outport  Port=165
  pne_brk_Axle4_right_torque : Outport  Port=166
  pne_brk_CompressorInlet_mdot : Outport  Port=167
  pne_brk_PowerBoost_massfracH2O : Outport  Port=168
  pne_brk_PowerBoost_pressure : Outport  Port=169
  pne_brk_PowerBoost_Temperature : Outport  Port=170
  pne_brk_TrailerAxle1_left_torque : Outport  Port=171
  pne_brk_TrailerAxle1_right_torque : Outport  Port=172
  pne_brk_TrailerAxle2_left_torque : Outport  Port=173
  pne_brk_TrailerAxle2_right_torque : Outport  Port=174
  pne_brk_TrailerAxle3_left_torque : Outport  Port=175
  pne_brk_TrailerAxle3_right_torque : Outport  Port=176
  pne_brk_Actual_Pressure_AL : Outport  Port=177
  pne_brk_Actual_Pressure_AR : Outport  Port=178
  pne_brk_Actual_Pressure_FA : Outport  Port=179
  pne_brk_Actual_Pressure_FOPB : Outport  Port=180
  pne_brk_Actual_Pressure_Front : Outport  Port=181
  pne_brk_Actual_Pressure_Rear : Outport  Port=182
  pne_brk_Actual_Pressure_RL : Outport  Port=183
  pne_brk_Actual_Pressure_RR : Outport  Port=184
  pne_brk_Actual_Pressure_TCV : Outport  Port=185
  pne_brk_AdditionalAxle_AxMo_left_rotVel : Outport  Port=186
  pne_brk_AdditionalAxle_AxMo_right_rotVel : Outport  Port=187
  pne_brk_AdditionalAxle_left_pAct : Outport  Port=188
  pne_brk_AdditionalAxle_left_rotVel : Outport  Port=189
  pne_brk_AdditionalAxle_right_pAct : Outport  Port=190
  pne_brk_AdditionalAxle_right_rotVel : Outport  Port=191
  pne_brk_Axle1_BrakingForce_at8p5bar : Outport  Port=192
  pne_brk_Axle1_left_Tinterior : Outport  Port=193
  pne_brk_Axle1_right_Tinterior : Outport  Port=194
  pne_brk_Axle1_torque_sns : Outport  Port=195
  pne_brk_Axle2_BrakingForce_at8p5bar : Outport  Port=196
  pne_brk_Axle2_left_Tinterior : Outport  Port=197
  pne_brk_Axle2_right_Tinterior : Outport  Port=198
  pne_brk_Axle2_torque_sns : Outport  Port=199
  pne_brk_Axle3_BrakingForce_at8p5bar : Outport  Port=200
  pne_brk_Axle3_left_Tinterior : Outport  Port=201
  pne_brk_Axle3_right_Tinterior : Outport  Port=202
  pne_brk_Axle3_torque_sns : Outport  Port=203
  pne_brk_Axle4_BrakingForce_at8p5bar : Outport  Port=204
  pne_brk_Axle4_left_Tinterior : Outport  Port=205
  pne_brk_Axle4_right_Tinterior : Outport  Port=206
  pne_brk_Axle4_torque_sns : Outport  Port=207
  pne_brk_BrkWearAALt : Outport  Port=208
  pne_brk_BrkWearAARt : Outport  Port=209
  pne_brk_BrkWearFA1Lt : Outport  Port=210
  pne_brk_BrkWearFA1Rt : Outport  Port=211
  pne_brk_BrkWearFA2Lt : Outport  Port=212
  pne_brk_BrkWearFA2Rt : Outport  Port=213
  pne_brk_BrkWearRA1Lt : Outport  Port=214
  pne_brk_BrkWearRA1Rt : Outport  Port=215
  pne_brk_BrkWearRA2Lt : Outport  Port=216
  pne_brk_BrkWearRA2Rt : Outport  Port=217
  pne_brk_CompON : Outport  Port=218
  pne_brk_FrontAxle_left_rotVel : Outport  Port=219
  pne_brk_FrontAxle_pAct : Outport  Port=220
  pne_brk_FrontAxle_right_rotVel : Outport  Port=221
  pne_brk_pRelPkBrk : Outport  Port=222
  pne_brk_RearAxle_left_pAct : Outport  Port=223
  pne_brk_RearAxle_left_rotVel : Outport  Port=224
  pne_brk_RearAxle_right_pAct : Outport  Port=225
  pne_brk_RearAxle_right_rotVel : Outport  Port=226
  pne_brk_reg_active : Outport  Port=227
  pne_brk_rotVel_al : Outport  Port=228
  pne_brk_rotVel_ar : Outport  Port=229
  pne_brk_rotVel_fl : Outport  Port=230
  pne_brk_rotVel_fr : Outport  Port=231
  pne_brk_rotVel_rl : Outport  Port=232
  pne_brk_rotVel_rr : Outport  Port=233
  pne_brk_rotVel_t1l : Outport  Port=234
  pne_brk_rotVel_t1r : Outport  Port=235
  pne_brk_rotVel_t2l : Outport  Port=236
  pne_brk_rotVel_t2r : Outport  Port=237
  pne_brk_rotVel_t3l : Outport  Port=238
  pne_brk_rotVel_t3r : Outport  Port=239
  pne_brk_TCV_pAct : Outport  Port=240
  pne_brk_Trailer_RV_Front_pAct : Outport  Port=241
  pne_brk_Trailer_RV_Rear_pAct : Outport  Port=242
  pne_brk_TrailerAxle1_BrakingForce_at8p5bar : Outport  Port=243
  pne_brk_TrailerAxle1_torque_sns : Outport  Port=244
  pne_brk_TrailerAxle2_BrakingForce_at8p5bar : Outport  Port=245
  pne_brk_TrailerAxle2_torque_sns : Outport  Port=246
  pne_brk_TrailerAxle3_BrakingForce_at8p5bar : Outport  Port=247
  pne_brk_TrailerAxle3_torque_sns : Outport  Port=248
  pne_brk_V1_pRel : Outport  Port=249
  pne_brk_V2_pRel : Outport  Port=250
  pne_brk_V4_pRel : Outport  Port=251
  pne_brk_V7_pRel : Outport  Port=252
  pne_brk_VTrailer_pRel : Outport  Port=253
  pne_brk_WetLvl_Cntr : Outport  Port=254
  pne_susp_A1_Le_Posn : Outport  Port=255
  pne_susp_A1_Ri_Posn : Outport  Port=256
  pne_susp_A2_Le_Posn : Outport  Port=257
  pne_susp_A2_Ri_Posn : Outport  Port=258
  pne_susp_A3_Le_Posn : Outport  Port=259
  pne_susp_A3_Ri_Posn : Outport  Port=260
  wires:
  pne_pne3d_generic_std_sf/260 -> pne_susp_A3_Ri_Posn/1  "pne_susp_A3_Ri_Posn"
  pne_pne3d_generic_std_sf/259 -> pne_susp_A3_Le_Posn/1  "pne_susp_A3_Le_Posn"
  pne_pne3d_generic_std_sf/258 -> pne_susp_A2_Ri_Posn/1  "pne_susp_A2_Ri_Posn"
  pne_pne3d_generic_std_sf/257 -> pne_susp_A2_Le_Posn/1  "pne_susp_A2_Le_Posn"
  pne_pne3d_generic_std_sf/256 -> pne_susp_A1_Ri_Posn/1  "pne_susp_A1_Ri_Posn"
  pne_pne3d_generic_std_sf/255 -> pne_susp_A1_Le_Posn/1  "pne_susp_A1_Le_Posn"
  pne_pne3d_generic_std_sf/254 -> pne_brk_WetLvl_Cntr/1  "pne_brk_WetLvl_Cntr"
  pne_pne3d_generic_std_sf/253 -> pne_brk_VTrailer_pRel/1  "pne_brk_VTrailer_pRel"
  pne_pne3d_generic_std_sf/252 -> pne_brk_V7_pRel/1  "pne_brk_V7_pRel"
  pne_pne3d_generic_std_sf/251 -> pne_brk_V4_pRel/1  "pne_brk_V4_pRel"
  pne_pne3d_generic_std_sf/250 -> pne_brk_V2_pRel/1  "pne_brk_V2_pRel"
  pne_pne3d_generic_std_sf/249 -> pne_brk_V1_pRel/1  "pne_brk_V1_pRel"
  pne_pne3d_generic_std_sf/248 -> pne_brk_TrailerAxle3_torque_sns/1  "pne_brk_TrailerAxle3_torque_sns"
  pne_pne3d_generic_std_sf/247 -> pne_brk_TrailerAxle3_BrakingForce_at8p5bar/1  "pne_brk_TrailerAxle3_BrakingForce_at8p5bar"
  pne_pne3d_generic_std_sf/246 -> pne_brk_TrailerAxle2_torque_sns/1  "pne_brk_TrailerAxle2_torque_sns"
  pne_pne3d_generic_std_sf/245 -> pne_brk_TrailerAxle2_BrakingForce_at8p5bar/1  "pne_brk_TrailerAxle2_BrakingForce_at8p5bar"
  pne_pne3d_generic_std_sf/244 -> pne_brk_TrailerAxle1_torque_sns/1  "pne_brk_TrailerAxle1_torque_sns"
  pne_pne3d_generic_std_sf/243 -> pne_brk_TrailerAxle1_BrakingForce_at8p5bar/1  "pne_brk_TrailerAxle1_BrakingForce_at8p5bar"
  pne_pne3d_generic_std_sf/242 -> pne_brk_Trailer_RV_Rear_pAct/1  "pne_brk_Trailer_RV_Rear_pAct"
  pne_pne3d_generic_std_sf/241 -> pne_brk_Trailer_RV_Front_pAct/1  "pne_brk_Trailer_RV_Front_pAct"
  pne_pne3d_generic_std_sf/240 -> pne_brk_TCV_pAct/1  "pne_brk_TCV_pAct"
  pne_pne3d_generic_std_sf/239 -> pne_brk_rotVel_t3r/1  "pne_brk_rotVel_t3r"
  pne_pne3d_generic_std_sf/238 -> pne_brk_rotVel_t3l/1  "pne_brk_rotVel_t3l"
  pne_pne3d_generic_std_sf/237 -> pne_brk_rotVel_t2r/1  "pne_brk_rotVel_t2r"
  pne_pne3d_generic_std_sf/236 -> pne_brk_rotVel_t2l/1  "pne_brk_rotVel_t2l"
  pne_pne3d_generic_std_sf/235 -> pne_brk_rotVel_t1r/1  "pne_brk_rotVel_t1r"
  pne_pne3d_generic_std_sf/234 -> pne_brk_rotVel_t1l/1  "pne_brk_rotVel_t1l"
  pne_pne3d_generic_std_sf/233 -> pne_brk_rotVel_rr/1  "pne_brk_rotVel_rr"
  pne_pne3d_generic_std_sf/232 -> pne_brk_rotVel_rl/1  "pne_brk_rotVel_rl"
  pne_pne3d_generic_std_sf/231 -> pne_brk_rotVel_fr/1  "pne_brk_rotVel_fr"
  pne_pne3d_generic_std_sf/230 -> pne_brk_rotVel_fl/1  "pne_brk_rotVel_fl"
  pne_pne3d_generic_std_sf/229 -> pne_brk_rotVel_ar/1  "pne_brk_rotVel_ar"
  pne_pne3d_generic_std_sf/228 -> pne_brk_rotVel_al/1  "pne_brk_rotVel_al"
  pne_pne3d_generic_std_sf/227 -> pne_brk_reg_active/1  "pne_brk_reg_active"
  pne_pne3d_generic_std_sf/226 -> pne_brk_RearAxle_right_rotVel/1  "pne_brk_RearAxle_right_rotVel"
  pne_pne3d_generic_std_sf/225 -> pne_brk_RearAxle_right_pAct/1  "pne_brk_RearAxle_right_pAct"
  pne_pne3d_generic_std_sf/224 -> pne_brk_RearAxle_left_rotVel/1  "pne_brk_RearAxle_left_rotVel"
  pne_pne3d_generic_std_sf/223 -> pne_brk_RearAxle_left_pAct/1  "pne_brk_RearAxle_left_pAct"
  pne_pne3d_generic_std_sf/222 -> pne_brk_pRelPkBrk/1  "pne_brk_pRelPkBrk"
  pne_pne3d_generic_std_sf/221 -> pne_brk_FrontAxle_right_rotVel/1  "pne_brk_FrontAxle_right_rotVel"
  pne_pne3d_generic_std_sf/220 -> pne_brk_FrontAxle_pAct/1  "pne_brk_FrontAxle_pAct"
  pne_pne3d_generic_std_sf/219 -> pne_brk_FrontAxle_left_rotVel/1  "pne_brk_FrontAxle_left_rotVel"
  pne_pne3d_generic_std_sf/218 -> pne_brk_CompON/1  "pne_brk_CompON"
  pne_pne3d_generic_std_sf/217 -> pne_brk_BrkWearRA2Rt/1  "pne_brk_BrkWearRA2Rt"
  pne_pne3d_generic_std_sf/216 -> pne_brk_BrkWearRA2Lt/1  "pne_brk_BrkWearRA2Lt"
  pne_pne3d_generic_std_sf/215 -> pne_brk_BrkWearRA1Rt/1  "pne_brk_BrkWearRA1Rt"
  pne_pne3d_generic_std_sf/214 -> pne_brk_BrkWearRA1Lt/1  "pne_brk_BrkWearRA1Lt"
  pne_pne3d_generic_std_sf/213 -> pne_brk_BrkWearFA2Rt/1  "pne_brk_BrkWearFA2Rt"
  pne_pne3d_generic_std_sf/212 -> pne_brk_BrkWearFA2Lt/1  "pne_brk_BrkWearFA2Lt"
  pne_pne3d_generic_std_sf/211 -> pne_brk_BrkWearFA1Rt/1  "pne_brk_BrkWearFA1Rt"
  pne_pne3d_generic_std_sf/210 -> pne_brk_BrkWearFA1Lt/1  "pne_brk_BrkWearFA1Lt"
  pne_pne3d_generic_std_sf/209 -> pne_brk_BrkWearAARt/1  "pne_brk_BrkWearAARt"
